simulink model "GIT_AUTO_Model_Example"  (R2019b)
settings: Solver=FixedStepDiscrete  StartTime=0.0  StopTime=10  FixedStep=0.01  RelTol=1e-3  EnableMultiTasking=on
InitFcn:
  | clear mex;
undefined symbols (not defined in the file): asbcbaseini_C, ibatini_C, k_icalpl_C, scsocini_C, stopengstmode_C, t_bmaxini_C, t_bminini_C, t_vminddstr_C, TSB_Coulomb_float, TSB_Dc_float, TSB_Pwr_float, TSB_R_float, TSB_Soc, TSB_Tbatt, TSB_Tbatt_float, TSB_value_float, TSB_Volt_float, v_bcini_C, v_bcmaxini_C
libraries: Utility_Block_Library x22, AMO_Block_Library x2
(part 4 of 5)

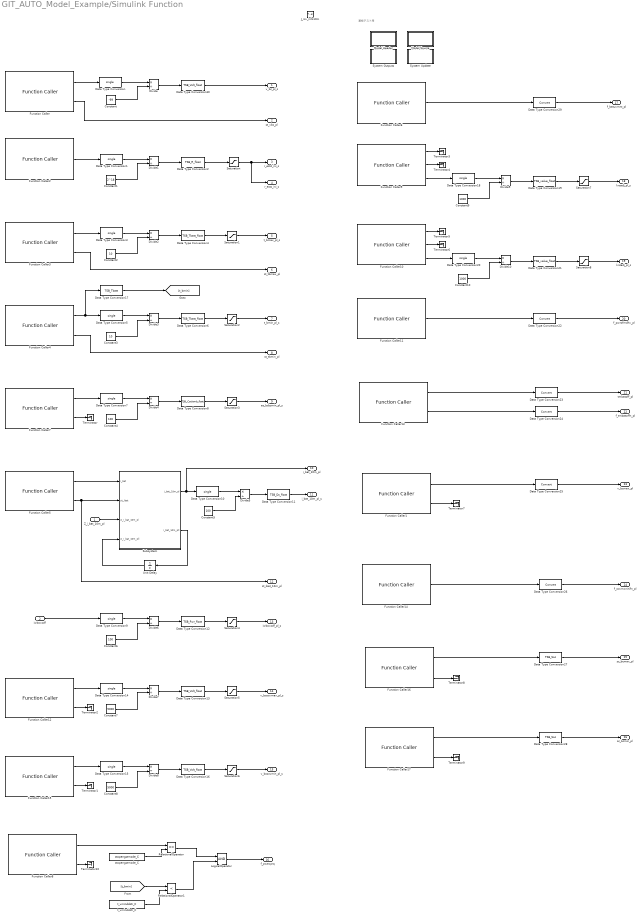
== system GIT_AUTO_Model_Example/Simulink Function ==
  note: 基板テスト用
  Z_i_bat_10m_pl : Inport  Tag=#AMO_Lib
      settings: AttributesFormatString=%<Tag>\n%<Description>\nSampleTime = %<SampleTime>
  iwboxcdf : Inport  Tag=#AMO_Lib  Port=2
      settings: AttributesFormatString=%<Tag>\n%<Description>\nSampleTime = %<SampleTime>
  J_rcv_info10m : TriggerPort  TriggerType=function-call  IsSimulinkFunction=on  FunctionName=J_rcv_info10m  VariantControl=(inherit)
  Constant : Constant  Tag=#AMO_Lib  Value=-99  OutDataTypeStr=single
      settings: AttributesFormatString=%<Tag>\nOutDataType = %<OutDataTypeStr>
  Constant1 : Constant  Tag=#AMO_Lib  Value=2^18  OutDataTypeStr=single
      settings: AttributesFormatString=%<Tag>\nOutDataType = %<OutDataTypeStr>
  Constant10 : Constant  Tag=#AMO_Lib  Value=1000  OutDataTypeStr=single
      settings: AttributesFormatString=%<Tag>\nOutDataType = %<OutDataTypeStr>
  Constant2 : Constant  Tag=#AMO_Lib  Value=10  OutDataTypeStr=single
      settings: AttributesFormatString=%<Tag>\nOutDataType = %<OutDataTypeStr>
  Constant3 : Constant  Tag=#AMO_Lib  Value=10  OutDataTypeStr=single
      settings: AttributesFormatString=%<Tag>\nOutDataType = %<OutDataTypeStr>
  Constant4 : Constant  Tag=#AMO_Lib  Value=100  OutDataTypeStr=single
      settings: AttributesFormatString=%<Tag>\nOutDataType = %<OutDataTypeStr>
  Constant5 : Constant  Tag=#AMO_Lib  Value=100  OutDataTypeStr=single
      settings: AttributesFormatString=%<Tag>\nOutDataType = %<OutDataTypeStr>
  Constant6 : Constant  Tag=#AMO_Lib  Value=100  OutDataTypeStr=single
      settings: AttributesFormatString=%<Tag>\nOutDataType = %<OutDataTypeStr>
  Constant7 : Constant  Tag=#AMO_Lib  Value=5000  OutDataTypeStr=single
      settings: AttributesFormatString=%<Tag>\nOutDataType = %<OutDataTypeStr>
  Constant8 : Constant  Tag=#AMO_Lib  Value=5000  OutDataTypeStr=single
      settings: AttributesFormatString=%<Tag>\nOutDataType = %<OutDataTypeStr>
  Constant9 : Constant  Tag=#AMO_Lib  Value=1000  OutDataTypeStr=single
      settings: AttributesFormatString=%<Tag>\nOutDataType = %<OutDataTypeStr>
  Data Type Conversion : DataTypeConversion  Tag=#AMO_Lib  OutMin=OutMin  OutMax=OutMax  OutDataTypeStr=single  ConvertRealWorld=Stored Integer (SI)  SampleTime=SampleTime  SaturateOnIntegerOverflow=on  RndMeth=Zero  mask{OutMin=[], OutMax=[], OutDataTypeStr=single, LockScale=off, ConvertRealWorld=Stored Integer (SI), RndMeth=Zero, SaturateOnIntegerOverflow=on, SampleTime=-1}
      mask prompts: OutMin "Simulink:blkprm_prompts:OutputDesignMin"; OutMax "Simulink:blkprm_prompts:OutputDesignMax"; OutDataTypeStr "Simulink:blkprm_prompts:OUTPUT_UNIFIEDDATATYPE"; LockScale "Simulink:blkprm_prompts:LockScale"; ConvertRealWorld "Simulink:blkprm_prompts:DtypeCnvInputOutputValue"; RndMeth "Simulink:blkprm_prompts:SPP_RndMeth_ID"; SaturateOnIntegerOverflow "Simulink:blkprm_prompts:AllBlksSaturate"; SampleTime "Simulink:blkprm_prompts:AllBlksSampleTime"
      mask help:
      | 入力を出力のデータ型とスケーリングに変換します。
      |
      | この変換には 2 つの目的があります。1 つは入力と出力の実際値を等しくすることです。もう 1 つは入力と出力の整数格納値を等しくすることです。オーバーフローと量子化誤差があると、この目的を完全に達成することができません。
      settings: AttributesFormatString=%<Tag>\nOutDataType = %<OutDataTypeStr>
      mask TypeOptions OutMin: OutMin
      mask TypeOptions OutMax: OutMax
      mask TypeOptions OutDataTypeStr: OutDataTypeStr
      mask TypeOptions LockScale: LockScale
      mask TypeOptions ConvertRealWorld: ConvertRealWorld
      mask TypeOptions RndMeth: RndMeth
      mask TypeOptions SaturateOnIntegerOverflow: SaturateOnIntegerOverflow
      mask TypeOptions SampleTime: SampleTime
      mask DialogControl OutMin Prompt: 出力の最小値:
      mask DialogControl OutMax Prompt: 出力の最大値:
      mask DialogControl OutDataTypeStr Prompt: 出力データ型:
      mask DialogControl LockScale Prompt: 固定小数点ツールによる変更に対して出力データ型の設定をロックする
      mask DialogControl ConvertRealWorld Prompt: 等価な値をもつ入力と出力:
      mask DialogControl RndMeth Prompt: 整数丸めモード:
      mask DialogControl SaturateOnIntegerOverflow Prompt: 整数オーバーフローで飽和
      mask DialogControl SampleTime Prompt: サンプル時間 (継承は -1):
  Data Type Conversion1 : DataTypeConversion  Tag=#AMO_Lib  OutMin=OutMin  OutMax=OutMax  OutDataTypeStr=single  ConvertRealWorld=Stored Integer (SI)  SampleTime=SampleTime  SaturateOnIntegerOverflow=on  RndMeth=Zero  mask{OutMin=[], OutMax=[], OutDataTypeStr=single, LockScale=off, ConvertRealWorld=Stored Integer (SI), RndMeth=Zero, SaturateOnIntegerOverflow=on, SampleTime=-1}
      mask prompts: OutMin "Simulink:blkprm_prompts:OutputDesignMin"; OutMax "Simulink:blkprm_prompts:OutputDesignMax"; OutDataTypeStr "Simulink:blkprm_prompts:OUTPUT_UNIFIEDDATATYPE"; LockScale "Simulink:blkprm_prompts:LockScale"; ConvertRealWorld "Simulink:blkprm_prompts:DtypeCnvInputOutputValue"; RndMeth "Simulink:blkprm_prompts:SPP_RndMeth_ID"; SaturateOnIntegerOverflow "Simulink:blkprm_prompts:AllBlksSaturate"; SampleTime "Simulink:blkprm_prompts:AllBlksSampleTime"
      mask help:
      | 入力を出力のデータ型とスケーリングに変換します。
      |
      | この変換には 2 つの目的があります。1 つは入力と出力の実際値を等しくすることです。もう 1 つは入力と出力の整数格納値を等しくすることです。オーバーフローと量子化誤差があると、この目的を完全に達成することができません。
      settings: AttributesFormatString=%<Tag>\nOutDataType = %<OutDataTypeStr>
      mask TypeOptions OutMin: OutMin
      mask TypeOptions OutMax: OutMax
      mask TypeOptions OutDataTypeStr: OutDataTypeStr
      mask TypeOptions LockScale: LockScale
      mask TypeOptions ConvertRealWorld: ConvertRealWorld
      mask TypeOptions RndMeth: RndMeth
      mask TypeOptions SaturateOnIntegerOverflow: SaturateOnIntegerOverflow
      mask TypeOptions SampleTime: SampleTime
      mask DialogControl OutMin Prompt: 出力の最小値:
      mask DialogControl OutMax Prompt: 出力の最大値:
      mask DialogControl OutDataTypeStr Prompt: 出力データ型:
      mask DialogControl LockScale Prompt: 固定小数点ツールによる変更に対して出力データ型の設定をロックする
      mask DialogControl ConvertRealWorld Prompt: 等価な値をもつ入力と出力:
      mask DialogControl RndMeth Prompt: 整数丸めモード:
      mask DialogControl SaturateOnIntegerOverflow Prompt: 整数オーバーフローで飽和
      mask DialogControl SampleTime Prompt: サンプル時間 (継承は -1):
  Data Type Conversion10 : DataTypeConversion  Tag=#AMO_Lib  OutMin=OutMin  OutMax=OutMax  OutDataTypeStr=single  ConvertRealWorld=Stored Integer (SI)  SampleTime=SampleTime  SaturateOnIntegerOverflow=on  RndMeth=Zero  mask{OutMin=[], OutMax=[], OutDataTypeStr=single, LockScale=off, ConvertRealWorld=Stored Integer (SI), RndMeth=Zero, SaturateOnIntegerOverflow=on, SampleTime=-1}
      mask prompts: OutMin "Simulink:blkprm_prompts:OutputDesignMin"; OutMax "Simulink:blkprm_prompts:OutputDesignMax"; OutDataTypeStr "Simulink:blkprm_prompts:OUTPUT_UNIFIEDDATATYPE"; LockScale "Simulink:blkprm_prompts:LockScale"; ConvertRealWorld "Simulink:blkprm_prompts:DtypeCnvInputOutputValue"; RndMeth "Simulink:blkprm_prompts:SPP_RndMeth_ID"; SaturateOnIntegerOverflow "Simulink:blkprm_prompts:AllBlksSaturate"; SampleTime "Simulink:blkprm_prompts:AllBlksSampleTime"
      mask help:
      | 入力を出力のデータ型とスケーリングに変換します。
      |
      | この変換には 2 つの目的があります。1 つは入力と出力の実際値を等しくすることです。もう 1 つは入力と出力の整数格納値を等しくすることです。オーバーフローと量子化誤差があると、この目的を完全に達成することができません。
      settings: AttributesFormatString=%<Tag>\nOutDataType = %<OutDataTypeStr>
      mask TypeOptions OutMin: OutMin
      mask TypeOptions OutMax: OutMax
      mask TypeOptions OutDataTypeStr: OutDataTypeStr
      mask TypeOptions LockScale: LockScale
      mask TypeOptions ConvertRealWorld: ConvertRealWorld
      mask TypeOptions RndMeth: RndMeth
      mask TypeOptions SaturateOnIntegerOverflow: SaturateOnIntegerOverflow
      mask TypeOptions SampleTime: SampleTime
      mask DialogControl OutMin Prompt: 出力の最小値:
      mask DialogControl OutMax Prompt: 出力の最大値:
      mask DialogControl OutDataTypeStr Prompt: 出力データ型:
      mask DialogControl LockScale Prompt: 固定小数点ツールによる変更に対して出力データ型の設定をロックする
      mask DialogControl ConvertRealWorld Prompt: 等価な値をもつ入力と出力:
      mask DialogControl RndMeth Prompt: 整数丸めモード:
      mask DialogControl SaturateOnIntegerOverflow Prompt: 整数オーバーフローで飽和
      mask DialogControl SampleTime Prompt: サンプル時間 (継承は -1):
  Data Type Conversion11 : DataTypeConversion  Tag=#AMO_Lib  OutMin=OutMin  OutMax=OutMax  OutDataTypeStr=TSB_Dc_float  SampleTime=SampleTime  SaturateOnIntegerOverflow=on  RndMeth=Zero  mask{OutMin=[], OutMax=[], OutDataTypeStr=TSB_Dc_float, LockScale=off, ConvertRealWorld=Real World Value (RWV), RndMeth=Zero, SaturateOnIntegerOverflow=on, SampleTime=-1}
      mask prompts: OutMin "Simulink:blkprm_prompts:OutputDesignMin"; OutMax "Simulink:blkprm_prompts:OutputDesignMax"; OutDataTypeStr "Simulink:blkprm_prompts:OUTPUT_UNIFIEDDATATYPE"; LockScale "Simulink:blkprm_prompts:LockScale"; ConvertRealWorld "Simulink:blkprm_prompts:DtypeCnvInputOutputValue"; RndMeth "Simulink:blkprm_prompts:SPP_RndMeth_ID"; SaturateOnIntegerOverflow "Simulink:blkprm_prompts:AllBlksSaturate"; SampleTime "Simulink:blkprm_prompts:AllBlksSampleTime"
      mask help:
      | 入力を出力のデータ型とスケーリングに変換します。
      |
      | この変換には 2 つの目的があります。1 つは入力と出力の実際値を等しくすることです。もう 1 つは入力と出力の整数格納値を等しくすることです。オーバーフローと量子化誤差があると、この目的を完全に達成することができません。
      settings: AttributesFormatString=%<Tag>\nOutDataType = %<OutDataTypeStr>
      mask TypeOptions OutMin: OutMin
      mask TypeOptions OutMax: OutMax
      mask TypeOptions OutDataTypeStr: OutDataTypeStr
      mask TypeOptions LockScale: LockScale
      mask TypeOptions ConvertRealWorld: ConvertRealWorld
      mask TypeOptions RndMeth: RndMeth
      mask TypeOptions SaturateOnIntegerOverflow: SaturateOnIntegerOverflow
      mask TypeOptions SampleTime: SampleTime
      mask DialogControl OutMin Prompt: 出力の最小値:
      mask DialogControl OutMax Prompt: 出力の最大値:
      mask DialogControl OutDataTypeStr Prompt: 出力データ型:
      mask DialogControl LockScale Prompt: 固定小数点ツールによる変更に対して出力データ型の設定をロックする
      mask DialogControl ConvertRealWorld Prompt: 等価な値をもつ入力と出力:
      mask DialogControl RndMeth Prompt: 整数丸めモード:
      mask DialogControl SaturateOnIntegerOverflow Prompt: 整数オーバーフローで飽和
      mask DialogControl SampleTime Prompt: サンプル時間 (継承は -1):
  Data Type Conversion12 : DataTypeConversion  Tag=#AMO_Lib  OutMin=OutMin  OutMax=OutMax  OutDataTypeStr=TSB_Pwr_float  SampleTime=SampleTime  SaturateOnIntegerOverflow=on  RndMeth=Zero  mask{OutMin=[], OutMax=[], OutDataTypeStr=TSB_Pwr_float, LockScale=off, ConvertRealWorld=Real World Value (RWV), RndMeth=Zero, SaturateOnIntegerOverflow=on, SampleTime=-1}
      mask prompts: OutMin "Simulink:blkprm_prompts:OutputDesignMin"; OutMax "Simulink:blkprm_prompts:OutputDesignMax"; OutDataTypeStr "Simulink:blkprm_prompts:OUTPUT_UNIFIEDDATATYPE"; LockScale "Simulink:blkprm_prompts:LockScale"; ConvertRealWorld "Simulink:blkprm_prompts:DtypeCnvInputOutputValue"; RndMeth "Simulink:blkprm_prompts:SPP_RndMeth_ID"; SaturateOnIntegerOverflow "Simulink:blkprm_prompts:AllBlksSaturate"; SampleTime "Simulink:blkprm_prompts:AllBlksSampleTime"
      mask help:
      | 入力を出力のデータ型とスケーリングに変換します。
      |
      | この変換には 2 つの目的があります。1 つは入力と出力の実際値を等しくすることです。もう 1 つは入力と出力の整数格納値を等しくすることです。オーバーフローと量子化誤差があると、この目的を完全に達成することができません。
      settings: AttributesFormatString=%<Tag>\nOutDataType = %<OutDataTypeStr>
      mask TypeOptions OutMin: OutMin
      mask TypeOptions OutMax: OutMax
      mask TypeOptions OutDataTypeStr: OutDataTypeStr
      mask TypeOptions LockScale: LockScale
      mask TypeOptions ConvertRealWorld: ConvertRealWorld
      mask TypeOptions RndMeth: RndMeth
      mask TypeOptions SaturateOnIntegerOverflow: SaturateOnIntegerOverflow
      mask TypeOptions SampleTime: SampleTime
      mask DialogControl OutMin Prompt: 出力の最小値:
      mask DialogControl OutMax Prompt: 出力の最大値:
      mask DialogControl OutDataTypeStr Prompt: 出力データ型:
      mask DialogControl LockScale Prompt: 固定小数点ツールによる変更に対して出力データ型の設定をロックする
      mask DialogControl ConvertRealWorld Prompt: 等価な値をもつ入力と出力:
      mask DialogControl RndMeth Prompt: 整数丸めモード:
      mask DialogControl SaturateOnIntegerOverflow Prompt: 整数オーバーフローで飽和
      mask DialogControl SampleTime Prompt: サンプル時間 (継承は -1):
  Data Type Conversion13 : DataTypeConversion  Tag=#AMO_Lib  OutMin=OutMin  OutMax=OutMax  OutDataTypeStr=TSB_Volt_float  SampleTime=SampleTime  SaturateOnIntegerOverflow=on  RndMeth=Zero  mask{OutMin=[], OutMax=[], OutDataTypeStr=TSB_Volt_float, LockScale=off, ConvertRealWorld=Real World Value (RWV), RndMeth=Zero, SaturateOnIntegerOverflow=on, SampleTime=-1}
      mask prompts: OutMin "Simulink:blkprm_prompts:OutputDesignMin"; OutMax "Simulink:blkprm_prompts:OutputDesignMax"; OutDataTypeStr "Simulink:blkprm_prompts:OUTPUT_UNIFIEDDATATYPE"; LockScale "Simulink:blkprm_prompts:LockScale"; ConvertRealWorld "Simulink:blkprm_prompts:DtypeCnvInputOutputValue"; RndMeth "Simulink:blkprm_prompts:SPP_RndMeth_ID"; SaturateOnIntegerOverflow "Simulink:blkprm_prompts:AllBlksSaturate"; SampleTime "Simulink:blkprm_prompts:AllBlksSampleTime"
      mask help:
      | 入力を出力のデータ型とスケーリングに変換します。
      |
      | この変換には 2 つの目的があります。1 つは入力と出力の実際値を等しくすることです。もう 1 つは入力と出力の整数格納値を等しくすることです。オーバーフローと量子化誤差があると、この目的を完全に達成することができません。
      settings: AttributesFormatString=%<Tag>\nOutDataType = %<OutDataTypeStr>
      mask TypeOptions OutMin: OutMin
      mask TypeOptions OutMax: OutMax
      mask TypeOptions OutDataTypeStr: OutDataTypeStr
      mask TypeOptions LockScale: LockScale
      mask TypeOptions ConvertRealWorld: ConvertRealWorld
      mask TypeOptions RndMeth: RndMeth
      mask TypeOptions SaturateOnIntegerOverflow: SaturateOnIntegerOverflow
      mask TypeOptions SampleTime: SampleTime
      mask DialogControl OutMin Prompt: 出力の最小値:
      mask DialogControl OutMax Prompt: 出力の最大値:
      mask DialogControl OutDataTypeStr Prompt: 出力データ型:
      mask DialogControl LockScale Prompt: 固定小数点ツールによる変更に対して出力データ型の設定をロックする
      mask DialogControl ConvertRealWorld Prompt: 等価な値をもつ入力と出力:
      mask DialogControl RndMeth Prompt: 整数丸めモード:
      mask DialogControl SaturateOnIntegerOverflow Prompt: 整数オーバーフローで飽和
      mask DialogControl SampleTime Prompt: サンプル時間 (継承は -1):
  Data Type Conversion14 : DataTypeConversion  Tag=#AMO_Lib  OutMin=OutMin  OutMax=OutMax  OutDataTypeStr=single  ConvertRealWorld=Stored Integer (SI)  SampleTime=SampleTime  SaturateOnIntegerOverflow=on  RndMeth=Zero  mask{OutMin=[], OutMax=[], OutDataTypeStr=single, LockScale=off, ConvertRealWorld=Stored Integer (SI), RndMeth=Zero, SaturateOnIntegerOverflow=on, SampleTime=-1}
      mask prompts: OutMin "Simulink:blkprm_prompts:OutputDesignMin"; OutMax "Simulink:blkprm_prompts:OutputDesignMax"; OutDataTypeStr "Simulink:blkprm_prompts:OUTPUT_UNIFIEDDATATYPE"; LockScale "Simulink:blkprm_prompts:LockScale"; ConvertRealWorld "Simulink:blkprm_prompts:DtypeCnvInputOutputValue"; RndMeth "Simulink:blkprm_prompts:SPP_RndMeth_ID"; SaturateOnIntegerOverflow "Simulink:blkprm_prompts:AllBlksSaturate"; SampleTime "Simulink:blkprm_prompts:AllBlksSampleTime"
      mask help:
      | 入力を出力のデータ型とスケーリングに変換します。
      |
      | この変換には 2 つの目的があります。1 つは入力と出力の実際値を等しくすることです。もう 1 つは入力と出力の整数格納値を等しくすることです。オーバーフローと量子化誤差があると、この目的を完全に達成することができません。
      settings: AttributesFormatString=%<Tag>\nOutDataType = %<OutDataTypeStr>
      mask TypeOptions OutMin: OutMin
      mask TypeOptions OutMax: OutMax
      mask TypeOptions OutDataTypeStr: OutDataTypeStr
      mask TypeOptions LockScale: LockScale
      mask TypeOptions ConvertRealWorld: ConvertRealWorld
      mask TypeOptions RndMeth: RndMeth
      mask TypeOptions SaturateOnIntegerOverflow: SaturateOnIntegerOverflow
      mask TypeOptions SampleTime: SampleTime
      mask DialogControl OutMin Prompt: 出力の最小値:
      mask DialogControl OutMax Prompt: 出力の最大値:
      mask DialogControl OutDataTypeStr Prompt: 出力データ型:
      mask DialogControl LockScale Prompt: 固定小数点ツールによる変更に対して出力データ型の設定をロックする
      mask DialogControl ConvertRealWorld Prompt: 等価な値をもつ入力と出力:
      mask DialogControl RndMeth Prompt: 整数丸めモード:
      mask DialogControl SaturateOnIntegerOverflow Prompt: 整数オーバーフローで飽和
      mask DialogControl SampleTime Prompt: サンプル時間 (継承は -1):
  Data Type Conversion15 : DataTypeConversion  Tag=#AMO_Lib  OutMin=OutMin  OutMax=OutMax  OutDataTypeStr=single  ConvertRealWorld=Stored Integer (SI)  SampleTime=SampleTime  SaturateOnIntegerOverflow=on  RndMeth=Zero  mask{OutMin=[], OutMax=[], OutDataTypeStr=single, LockScale=off, ConvertRealWorld=Stored Integer (SI), RndMeth=Zero, SaturateOnIntegerOverflow=on, SampleTime=-1}
      mask prompts: OutMin "Simulink:blkprm_prompts:OutputDesignMin"; OutMax "Simulink:blkprm_prompts:OutputDesignMax"; OutDataTypeStr "Simulink:blkprm_prompts:OUTPUT_UNIFIEDDATATYPE"; LockScale "Simulink:blkprm_prompts:LockScale"; ConvertRealWorld "Simulink:blkprm_prompts:DtypeCnvInputOutputValue"; RndMeth "Simulink:blkprm_prompts:SPP_RndMeth_ID"; SaturateOnIntegerOverflow "Simulink:blkprm_prompts:AllBlksSaturate"; SampleTime "Simulink:blkprm_prompts:AllBlksSampleTime"
      mask help:
      | 入力を出力のデータ型とスケーリングに変換します。
      |
      | この変換には 2 つの目的があります。1 つは入力と出力の実際値を等しくすることです。もう 1 つは入力と出力の整数格納値を等しくすることです。オーバーフローと量子化誤差があると、この目的を完全に達成することができません。
      settings: AttributesFormatString=%<Tag>\nOutDataType = %<OutDataTypeStr>
      mask TypeOptions OutMin: OutMin
      mask TypeOptions OutMax: OutMax
      mask TypeOptions OutDataTypeStr: OutDataTypeStr
      mask TypeOptions LockScale: LockScale
      mask TypeOptions ConvertRealWorld: ConvertRealWorld
      mask TypeOptions RndMeth: RndMeth
      mask TypeOptions SaturateOnIntegerOverflow: SaturateOnIntegerOverflow
      mask TypeOptions SampleTime: SampleTime
      mask DialogControl OutMin Prompt: 出力の最小値:
      mask DialogControl OutMax Prompt: 出力の最大値:
      mask DialogControl OutDataTypeStr Prompt: 出力データ型:
      mask DialogControl LockScale Prompt: 固定小数点ツールによる変更に対して出力データ型の設定をロックする
      mask DialogControl ConvertRealWorld Prompt: 等価な値をもつ入力と出力:
      mask DialogControl RndMeth Prompt: 整数丸めモード:
      mask DialogControl SaturateOnIntegerOverflow Prompt: 整数オーバーフローで飽和
      mask DialogControl SampleTime Prompt: サンプル時間 (継承は -1):
  Data Type Conversion16 : DataTypeConversion  Tag=#AMO_Lib  OutMin=OutMin  OutMax=OutMax  OutDataTypeStr=TSB_Volt_float  SampleTime=SampleTime  SaturateOnIntegerOverflow=on  RndMeth=Zero  mask{OutMin=[], OutMax=[], OutDataTypeStr=TSB_Volt_float, LockScale=off, ConvertRealWorld=Real World Value (RWV), RndMeth=Zero, SaturateOnIntegerOverflow=on, SampleTime=-1}
      mask prompts: OutMin "Simulink:blkprm_prompts:OutputDesignMin"; OutMax "Simulink:blkprm_prompts:OutputDesignMax"; OutDataTypeStr "Simulink:blkprm_prompts:OUTPUT_UNIFIEDDATATYPE"; LockScale "Simulink:blkprm_prompts:LockScale"; ConvertRealWorld "Simulink:blkprm_prompts:DtypeCnvInputOutputValue"; RndMeth "Simulink:blkprm_prompts:SPP_RndMeth_ID"; SaturateOnIntegerOverflow "Simulink:blkprm_prompts:AllBlksSaturate"; SampleTime "Simulink:blkprm_prompts:AllBlksSampleTime"
      mask help:
      | 入力を出力のデータ型とスケーリングに変換します。
      |
      | この変換には 2 つの目的があります。1 つは入力と出力の実際値を等しくすることです。もう 1 つは入力と出力の整数格納値を等しくすることです。オーバーフローと量子化誤差があると、この目的を完全に達成することができません。
      settings: AttributesFormatString=%<Tag>\nOutDataType = %<OutDataTypeStr>
      mask TypeOptions OutMin: OutMin
      mask TypeOptions OutMax: OutMax
      mask TypeOptions OutDataTypeStr: OutDataTypeStr
      mask TypeOptions LockScale: LockScale
      mask TypeOptions ConvertRealWorld: ConvertRealWorld
      mask TypeOptions RndMeth: RndMeth
      mask TypeOptions SaturateOnIntegerOverflow: SaturateOnIntegerOverflow
      mask TypeOptions SampleTime: SampleTime
      mask DialogControl OutMin Prompt: 出力の最小値:
      mask DialogControl OutMax Prompt: 出力の最大値:
      mask DialogControl OutDataTypeStr Prompt: 出力データ型:
      mask DialogControl LockScale Prompt: 固定小数点ツールによる変更に対して出力データ型の設定をロックする
      mask DialogControl ConvertRealWorld Prompt: 等価な値をもつ入力と出力:
      mask DialogControl RndMeth Prompt: 整数丸めモード:
      mask DialogControl SaturateOnIntegerOverflow Prompt: 整数オーバーフローで飽和
      mask DialogControl SampleTime Prompt: サンプル時間 (継承は -1):
  Data Type Conversion17 : DataTypeConversion  Tag=#AMO_Lib  OutMin=OutMin  OutMax=OutMax  OutDataTypeStr=TSB_Tbatt  ConvertRealWorld=Stored Integer (SI)  SampleTime=SampleTime  SaturateOnIntegerOverflow=on  RndMeth=Zero  mask{OutMin=[], OutMax=[], OutDataTypeStr=TSB_Tbatt, LockScale=off, ConvertRealWorld=Stored Integer (SI), RndMeth=Zero, SaturateOnIntegerOverflow=on, SampleTime=-1}
      mask prompts: OutMin "Simulink:blkprm_prompts:OutputDesignMin"; OutMax "Simulink:blkprm_prompts:OutputDesignMax"; OutDataTypeStr "Simulink:blkprm_prompts:OUTPUT_UNIFIEDDATATYPE"; LockScale "Simulink:blkprm_prompts:LockScale"; ConvertRealWorld "Simulink:blkprm_prompts:DtypeCnvInputOutputValue"; RndMeth "Simulink:blkprm_prompts:SPP_RndMeth_ID"; SaturateOnIntegerOverflow "Simulink:blkprm_prompts:AllBlksSaturate"; SampleTime "Simulink:blkprm_prompts:AllBlksSampleTime"
      mask help:
      | 入力を出力のデータ型とスケーリングに変換します。
      |
      | この変換には 2 つの目的があります。1 つは入力と出力の実際値を等しくすることです。もう 1 つは入力と出力の整数格納値を等しくすることです。オーバーフローと量子化誤差があると、この目的を完全に達成することができません。
      settings: AttributesFormatString=%<Tag>\nOutDataType = %<OutDataTypeStr>
      mask TypeOptions OutMin: OutMin
      mask TypeOptions OutMax: OutMax
      mask TypeOptions OutDataTypeStr: OutDataTypeStr
      mask TypeOptions LockScale: LockScale
      mask TypeOptions ConvertRealWorld: ConvertRealWorld
      mask TypeOptions RndMeth: RndMeth
      mask TypeOptions SaturateOnIntegerOverflow: SaturateOnIntegerOverflow
      mask TypeOptions SampleTime: SampleTime
      mask DialogControl OutMin Prompt: 出力の最小値:
      mask DialogControl OutMax Prompt: 出力の最大値:
      mask DialogControl OutDataTypeStr Prompt: 出力データ型:
      mask DialogControl LockScale Prompt: 固定小数点ツールによる変更に対して出力データ型の設定をロックする
      mask DialogControl ConvertRealWorld Prompt: 等価な値をもつ入力と出力:
      mask DialogControl RndMeth Prompt: 整数丸めモード:
      mask DialogControl SaturateOnIntegerOverflow Prompt: 整数オーバーフローで飽和
      mask DialogControl SampleTime Prompt: サンプル時間 (継承は -1):
  Data Type Conversion18 : DataTypeConversion  Tag=#AMO_Lib  OutMin=OutMin  OutMax=OutMax  OutDataTypeStr=single  ConvertRealWorld=Stored Integer (SI)  SampleTime=SampleTime  SaturateOnIntegerOverflow=on  RndMeth=Zero  mask{OutMin=[], OutMax=[], OutDataTypeStr=single, LockScale=off, ConvertRealWorld=Stored Integer (SI), RndMeth=Zero, SaturateOnIntegerOverflow=on, SampleTime=-1}
      mask prompts: OutMin "Simulink:blkprm_prompts:OutputDesignMin"; OutMax "Simulink:blkprm_prompts:OutputDesignMax"; OutDataTypeStr "Simulink:blkprm_prompts:OUTPUT_UNIFIEDDATATYPE"; LockScale "Simulink:blkprm_prompts:LockScale"; ConvertRealWorld "Simulink:blkprm_prompts:DtypeCnvInputOutputValue"; RndMeth "Simulink:blkprm_prompts:SPP_RndMeth_ID"; SaturateOnIntegerOverflow "Simulink:blkprm_prompts:AllBlksSaturate"; SampleTime "Simulink:blkprm_prompts:AllBlksSampleTime"
      mask help:
      | 入力を出力のデータ型とスケーリングに変換します。
      |
      | この変換には 2 つの目的があります。1 つは入力と出力の実際値を等しくすることです。もう 1 つは入力と出力の整数格納値を等しくすることです。オーバーフローと量子化誤差があると、この目的を完全に達成することができません。
      settings: AttributesFormatString=%<Tag>\nOutDataType = %<OutDataTypeStr>
      mask TypeOptions OutMin: OutMin
      mask TypeOptions OutMax: OutMax
      mask TypeOptions OutDataTypeStr: OutDataTypeStr
      mask TypeOptions LockScale: LockScale
      mask TypeOptions ConvertRealWorld: ConvertRealWorld
      mask TypeOptions RndMeth: RndMeth
      mask TypeOptions SaturateOnIntegerOverflow: SaturateOnIntegerOverflow
      mask TypeOptions SampleTime: SampleTime
      mask DialogControl OutMin Prompt: 出力の最小値:
      mask DialogControl OutMax Prompt: 出力の最大値:
      mask DialogControl OutDataTypeStr Prompt: 出力データ型:
      mask DialogControl LockScale Prompt: 固定小数点ツールによる変更に対して出力データ型の設定をロックする
      mask DialogControl ConvertRealWorld Prompt: 等価な値をもつ入力と出力:
      mask DialogControl RndMeth Prompt: 整数丸めモード:
      mask DialogControl SaturateOnIntegerOverflow Prompt: 整数オーバーフローで飽和
      mask DialogControl SampleTime Prompt: サンプル時間 (継承は -1):
  Data Type Conversion19 : DataTypeConversion  Tag=#AMO_Lib  OutMin=OutMin  OutMax=OutMax  OutDataTypeStr=TSB_value_float  SampleTime=SampleTime  SaturateOnIntegerOverflow=on  RndMeth=Zero  mask{OutMin=[], OutMax=[], OutDataTypeStr=TSB_value_float, LockScale=off, ConvertRealWorld=Real World Value (RWV), RndMeth=Zero, SaturateOnIntegerOverflow=on, SampleTime=-1}
      mask prompts: OutMin "Simulink:blkprm_prompts:OutputDesignMin"; OutMax "Simulink:blkprm_prompts:OutputDesignMax"; OutDataTypeStr "Simulink:blkprm_prompts:OUTPUT_UNIFIEDDATATYPE"; LockScale "Simulink:blkprm_prompts:LockScale"; ConvertRealWorld "Simulink:blkprm_prompts:DtypeCnvInputOutputValue"; RndMeth "Simulink:blkprm_prompts:SPP_RndMeth_ID"; SaturateOnIntegerOverflow "Simulink:blkprm_prompts:AllBlksSaturate"; SampleTime "Simulink:blkprm_prompts:AllBlksSampleTime"
      mask help:
      | 入力を出力のデータ型とスケーリングに変換します。
      |
      | この変換には 2 つの目的があります。1 つは入力と出力の実際値を等しくすることです。もう 1 つは入力と出力の整数格納値を等しくすることです。オーバーフローと量子化誤差があると、この目的を完全に達成することができません。
      settings: AttributesFormatString=%<Tag>\nOutDataType = %<OutDataTypeStr>
      mask TypeOptions OutMin: OutMin
      mask TypeOptions OutMax: OutMax
      mask TypeOptions OutDataTypeStr: OutDataTypeStr
      mask TypeOptions LockScale: LockScale
      mask TypeOptions ConvertRealWorld: ConvertRealWorld
      mask TypeOptions RndMeth: RndMeth
      mask TypeOptions SaturateOnIntegerOverflow: SaturateOnIntegerOverflow
      mask TypeOptions SampleTime: SampleTime
      mask DialogControl OutMin Prompt: 出力の最小値:
      mask DialogControl OutMax Prompt: 出力の最大値:
      mask DialogControl OutDataTypeStr Prompt: 出力データ型:
      mask DialogControl LockScale Prompt: 固定小数点ツールによる変更に対して出力データ型の設定をロックする
      mask DialogControl ConvertRealWorld Prompt: 等価な値をもつ入力と出力:
      mask DialogControl RndMeth Prompt: 整数丸めモード:
      mask DialogControl SaturateOnIntegerOverflow Prompt: 整数オーバーフローで飽和
      mask DialogControl SampleTime Prompt: サンプル時間 (継承は -1):
  Data Type Conversion2 : DataTypeConversion  Tag=#AMO_Lib  OutMin=OutMin  OutMax=OutMax  OutDataTypeStr=TSB_R_float  SampleTime=SampleTime  SaturateOnIntegerOverflow=on  RndMeth=Zero  mask{OutMin=[], OutMax=[], OutDataTypeStr=TSB_R_float, LockScale=off, ConvertRealWorld=Real World Value (RWV), RndMeth=Zero, SaturateOnIntegerOverflow=on, SampleTime=-1}
      mask prompts: OutMin "Simulink:blkprm_prompts:OutputDesignMin"; OutMax "Simulink:blkprm_prompts:OutputDesignMax"; OutDataTypeStr "Simulink:blkprm_prompts:OUTPUT_UNIFIEDDATATYPE"; LockScale "Simulink:blkprm_prompts:LockScale"; ConvertRealWorld "Simulink:blkprm_prompts:DtypeCnvInputOutputValue"; RndMeth "Simulink:blkprm_prompts:SPP_RndMeth_ID"; SaturateOnIntegerOverflow "Simulink:blkprm_prompts:AllBlksSaturate"; SampleTime "Simulink:blkprm_prompts:AllBlksSampleTime"
      mask help:
      | 入力を出力のデータ型とスケーリングに変換します。
      |
      | この変換には 2 つの目的があります。1 つは入力と出力の実際値を等しくすることです。もう 1 つは入力と出力の整数格納値を等しくすることです。オーバーフローと量子化誤差があると、この目的を完全に達成することができません。
      settings: AttributesFormatString=%<Tag>\nOutDataType = %<OutDataTypeStr>
      mask TypeOptions OutMin: OutMin
      mask TypeOptions OutMax: OutMax
      mask TypeOptions OutDataTypeStr: OutDataTypeStr
      mask TypeOptions LockScale: LockScale
      mask TypeOptions ConvertRealWorld: ConvertRealWorld
      mask TypeOptions RndMeth: RndMeth
      mask TypeOptions SaturateOnIntegerOverflow: SaturateOnIntegerOverflow
      mask TypeOptions SampleTime: SampleTime
      mask DialogControl OutMin Prompt: 出力の最小値:
      mask DialogControl OutMax Prompt: 出力の最大値:
      mask DialogControl OutDataTypeStr Prompt: 出力データ型:
      mask DialogControl LockScale Prompt: 固定小数点ツールによる変更に対して出力データ型の設定をロックする
      mask DialogControl ConvertRealWorld Prompt: 等価な値をもつ入力と出力:
      mask DialogControl RndMeth Prompt: 整数丸めモード:
      mask DialogControl SaturateOnIntegerOverflow Prompt: 整数オーバーフローで飽和
      mask DialogControl SampleTime Prompt: サンプル時間 (継承は -1):
  Data Type Conversion20 : DataTypeConversion  Tag=#AMO_Lib  OutMin=OutMin  OutMax=OutMax  OutDataTypeStr=single  ConvertRealWorld=Stored Integer (SI)  SampleTime=SampleTime  SaturateOnIntegerOverflow=on  RndMeth=Zero  mask{OutMin=[], OutMax=[], OutDataTypeStr=single, LockScale=off, ConvertRealWorld=Stored Integer (SI), RndMeth=Zero, SaturateOnIntegerOverflow=on, SampleTime=-1}
      mask prompts: OutMin "Simulink:blkprm_prompts:OutputDesignMin"; OutMax "Simulink:blkprm_prompts:OutputDesignMax"; OutDataTypeStr "Simulink:blkprm_prompts:OUTPUT_UNIFIEDDATATYPE"; LockScale "Simulink:blkprm_prompts:LockScale"; ConvertRealWorld "Simulink:blkprm_prompts:DtypeCnvInputOutputValue"; RndMeth "Simulink:blkprm_prompts:SPP_RndMeth_ID"; SaturateOnIntegerOverflow "Simulink:blkprm_prompts:AllBlksSaturate"; SampleTime "Simulink:blkprm_prompts:AllBlksSampleTime"
      mask help:
      | 入力を出力のデータ型とスケーリングに変換します。
      |
      | この変換には 2 つの目的があります。1 つは入力と出力の実際値を等しくすることです。もう 1 つは入力と出力の整数格納値を等しくすることです。オーバーフローと量子化誤差があると、この目的を完全に達成することができません。
      settings: AttributesFormatString=%<Tag>\nOutDataType = %<OutDataTypeStr>
      mask TypeOptions OutMin: OutMin
      mask TypeOptions OutMax: OutMax
      mask TypeOptions OutDataTypeStr: OutDataTypeStr
      mask TypeOptions LockScale: LockScale
      mask TypeOptions ConvertRealWorld: ConvertRealWorld
      mask TypeOptions RndMeth: RndMeth
      mask TypeOptions SaturateOnIntegerOverflow: SaturateOnIntegerOverflow
      mask TypeOptions SampleTime: SampleTime
      mask DialogControl OutMin Prompt: 出力の最小値:
      mask DialogControl OutMax Prompt: 出力の最大値:
      mask DialogControl OutDataTypeStr Prompt: 出力データ型:
      mask DialogControl LockScale Prompt: 固定小数点ツールによる変更に対して出力データ型の設定をロックする
      mask DialogControl ConvertRealWorld Prompt: 等価な値をもつ入力と出力:
      mask DialogControl RndMeth Prompt: 整数丸めモード:
      mask DialogControl SaturateOnIntegerOverflow Prompt: 整数オーバーフローで飽和
      mask DialogControl SampleTime Prompt: サンプル時間 (継承は -1):
  Data Type Conversion21 : DataTypeConversion  Tag=#AMO_Lib  OutMin=OutMin  OutMax=OutMax  OutDataTypeStr=TSB_value_float  SampleTime=SampleTime  SaturateOnIntegerOverflow=on  RndMeth=Zero  mask{OutMin=[], OutMax=[], OutDataTypeStr=TSB_value_float, LockScale=off, ConvertRealWorld=Real World Value (RWV), RndMeth=Zero, SaturateOnIntegerOverflow=on, SampleTime=-1}
      mask prompts: OutMin "Simulink:blkprm_prompts:OutputDesignMin"; OutMax "Simulink:blkprm_prompts:OutputDesignMax"; OutDataTypeStr "Simulink:blkprm_prompts:OUTPUT_UNIFIEDDATATYPE"; LockScale "Simulink:blkprm_prompts:LockScale"; ConvertRealWorld "Simulink:blkprm_prompts:DtypeCnvInputOutputValue"; RndMeth "Simulink:blkprm_prompts:SPP_RndMeth_ID"; SaturateOnIntegerOverflow "Simulink:blkprm_prompts:AllBlksSaturate"; SampleTime "Simulink:blkprm_prompts:AllBlksSampleTime"
      mask help:
      | 入力を出力のデータ型とスケーリングに変換します。
      |
      | この変換には 2 つの目的があります。1 つは入力と出力の実際値を等しくすることです。もう 1 つは入力と出力の整数格納値を等しくすることです。オーバーフローと量子化誤差があると、この目的を完全に達成することができません。
      settings: AttributesFormatString=%<Tag>\nOutDataType = %<OutDataTypeStr>
      mask TypeOptions OutMin: OutMin
      mask TypeOptions OutMax: OutMax
      mask TypeOptions OutDataTypeStr: OutDataTypeStr
      mask TypeOptions LockScale: LockScale
      mask TypeOptions ConvertRealWorld: ConvertRealWorld
      mask TypeOptions RndMeth: RndMeth
      mask TypeOptions SaturateOnIntegerOverflow: SaturateOnIntegerOverflow
      mask TypeOptions SampleTime: SampleTime
      mask DialogControl OutMin Prompt: 出力の最小値:
      mask DialogControl OutMax Prompt: 出力の最大値:
      mask DialogControl OutDataTypeStr Prompt: 出力データ型:
      mask DialogControl LockScale Prompt: 固定小数点ツールによる変更に対して出力データ型の設定をロックする
      mask DialogControl ConvertRealWorld Prompt: 等価な値をもつ入力と出力:
      mask DialogControl RndMeth Prompt: 整数丸めモード:
      mask DialogControl SaturateOnIntegerOverflow Prompt: 整数オーバーフローで飽和
      mask DialogControl SampleTime Prompt: サンプル時間 (継承は -1):
  Data Type Conversion22 : DataTypeConversion  Tag=#AMO_Lib  OutMin=OutMin  OutMax=OutMax  SampleTime=SampleTime  SaturateOnIntegerOverflow=on  RndMeth=Zero  mask{OutMin=[], OutMax=[], OutDataTypeStr=Inherit: Inherit via back propagation, LockScale=off, ConvertRealWorld=Real World Value (RWV), RndMeth=Zero, SaturateOnIntegerOverflow=on, SampleTime=-1}
      mask prompts: OutMin "Simulink:blkprm_prompts:OutputDesignMin"; OutMax "Simulink:blkprm_prompts:OutputDesignMax"; OutDataTypeStr "Simulink:blkprm_prompts:OUTPUT_UNIFIEDDATATYPE"; LockScale "Simulink:blkprm_prompts:LockScale"; ConvertRealWorld "Simulink:blkprm_prompts:DtypeCnvInputOutputValue"; RndMeth "Simulink:blkprm_prompts:SPP_RndMeth_ID"; SaturateOnIntegerOverflow "Simulink:blkprm_prompts:AllBlksSaturate"; SampleTime "Simulink:blkprm_prompts:AllBlksSampleTime"
      mask help:
      | 入力を出力のデータ型とスケーリングに変換します。
      |
      | この変換には 2 つの目的があります。1 つは入力と出力の実際値を等しくすることです。もう 1 つは入力と出力の整数格納値を等しくすることです。オーバーフローと量子化誤差があると、この目的を完全に達成することができません。
      settings: AttributesFormatString=%<Tag>\nOutDataType = %<OutDataTypeStr>
      mask TypeOptions OutMin: OutMin
      mask TypeOptions OutMax: OutMax
      mask TypeOptions OutDataTypeStr: OutDataTypeStr
      mask TypeOptions LockScale: LockScale
      mask TypeOptions ConvertRealWorld: ConvertRealWorld
      mask TypeOptions RndMeth: RndMeth
      mask TypeOptions SaturateOnIntegerOverflow: SaturateOnIntegerOverflow
      mask TypeOptions SampleTime: SampleTime
      mask DialogControl OutMin Prompt: 出力の最小値:
      mask DialogControl OutMax Prompt: 出力の最大値:
      mask DialogControl OutDataTypeStr Prompt: 出力データ型:
      mask DialogControl LockScale Prompt: 固定小数点ツールによる変更に対して出力データ型の設定をロックする
      mask DialogControl ConvertRealWorld Prompt: 等価な値をもつ入力と出力:
      mask DialogControl RndMeth Prompt: 整数丸めモード:
      mask DialogControl SaturateOnIntegerOverflow Prompt: 整数オーバーフローで飽和
      mask DialogControl SampleTime Prompt: サンプル時間 (継承は -1):
  Data Type Conversion23 : DataTypeConversion  Tag=#AMO_Lib  OutMin=OutMin  OutMax=OutMax  SampleTime=SampleTime  SaturateOnIntegerOverflow=on  RndMeth=Zero  mask{OutMin=[], OutMax=[], OutDataTypeStr=Inherit: Inherit via back propagation, LockScale=off, ConvertRealWorld=Real World Value (RWV), RndMeth=Zero, SaturateOnIntegerOverflow=on, SampleTime=-1}
      mask prompts: OutMin "Simulink:blkprm_prompts:OutputDesignMin"; OutMax "Simulink:blkprm_prompts:OutputDesignMax"; OutDataTypeStr "Simulink:blkprm_prompts:OUTPUT_UNIFIEDDATATYPE"; LockScale "Simulink:blkprm_prompts:LockScale"; ConvertRealWorld "Simulink:blkprm_prompts:DtypeCnvInputOutputValue"; RndMeth "Simulink:blkprm_prompts:SPP_RndMeth_ID"; SaturateOnIntegerOverflow "Simulink:blkprm_prompts:AllBlksSaturate"; SampleTime "Simulink:blkprm_prompts:AllBlksSampleTime"
      mask help:
      | 入力を出力のデータ型とスケーリングに変換します。
      |
      | この変換には 2 つの目的があります。1 つは入力と出力の実際値を等しくすることです。もう 1 つは入力と出力の整数格納値を等しくすることです。オーバーフローと量子化誤差があると、この目的を完全に達成することができません。
      settings: AttributesFormatString=%<Tag>\nOutDataType = %<OutDataTypeStr>
      mask TypeOptions OutMin: OutMin
      mask TypeOptions OutMax: OutMax
      mask TypeOptions OutDataTypeStr: OutDataTypeStr
      mask TypeOptions LockScale: LockScale
      mask TypeOptions ConvertRealWorld: ConvertRealWorld
      mask TypeOptions RndMeth: RndMeth
      mask TypeOptions SaturateOnIntegerOverflow: SaturateOnIntegerOverflow
      mask TypeOptions SampleTime: SampleTime
      mask DialogControl OutMin Prompt: 出力の最小値:
      mask DialogControl OutMax Prompt: 出力の最大値:
      mask DialogControl OutDataTypeStr Prompt: 出力データ型:
      mask DialogControl LockScale Prompt: 固定小数点ツールによる変更に対して出力データ型の設定をロックする
      mask DialogControl ConvertRealWorld Prompt: 等価な値をもつ入力と出力:
      mask DialogControl RndMeth Prompt: 整数丸めモード:
      mask DialogControl SaturateOnIntegerOverflow Prompt: 整数オーバーフローで飽和
      mask DialogControl SampleTime Prompt: サンプル時間 (継承は -1):
  Data Type Conversion24 : DataTypeConversion  Tag=#AMO_Lib  OutMin=OutMin  OutMax=OutMax  SampleTime=SampleTime  SaturateOnIntegerOverflow=on  RndMeth=Zero  mask{OutMin=[], OutMax=[], OutDataTypeStr=Inherit: Inherit via back propagation, LockScale=off, ConvertRealWorld=Real World Value (RWV), RndMeth=Zero, SaturateOnIntegerOverflow=on, SampleTime=-1}
      mask prompts: OutMin "Simulink:blkprm_prompts:OutputDesignMin"; OutMax "Simulink:blkprm_prompts:OutputDesignMax"; OutDataTypeStr "Simulink:blkprm_prompts:OUTPUT_UNIFIEDDATATYPE"; LockScale "Simulink:blkprm_prompts:LockScale"; ConvertRealWorld "Simulink:blkprm_prompts:DtypeCnvInputOutputValue"; RndMeth "Simulink:blkprm_prompts:SPP_RndMeth_ID"; SaturateOnIntegerOverflow "Simulink:blkprm_prompts:AllBlksSaturate"; SampleTime "Simulink:blkprm_prompts:AllBlksSampleTime"
      mask help:
      | 入力を出力のデータ型とスケーリングに変換します。
      |
      | この変換には 2 つの目的があります。1 つは入力と出力の実際値を等しくすることです。もう 1 つは入力と出力の整数格納値を等しくすることです。オーバーフローと量子化誤差があると、この目的を完全に達成することができません。
      settings: AttributesFormatString=%<Tag>\nOutDataType = %<OutDataTypeStr>
      mask TypeOptions OutMin: OutMin
      mask TypeOptions OutMax: OutMax
      mask TypeOptions OutDataTypeStr: OutDataTypeStr
      mask TypeOptions LockScale: LockScale
      mask TypeOptions ConvertRealWorld: ConvertRealWorld
      mask TypeOptions RndMeth: RndMeth
      mask TypeOptions SaturateOnIntegerOverflow: SaturateOnIntegerOverflow
      mask TypeOptions SampleTime: SampleTime
      mask DialogControl OutMin Prompt: 出力の最小値:
      mask DialogControl OutMax Prompt: 出力の最大値:
      mask DialogControl OutDataTypeStr Prompt: 出力データ型:
      mask DialogControl LockScale Prompt: 固定小数点ツールによる変更に対して出力データ型の設定をロックする
      mask DialogControl ConvertRealWorld Prompt: 等価な値をもつ入力と出力:
      mask DialogControl RndMeth Prompt: 整数丸めモード:
      mask DialogControl SaturateOnIntegerOverflow Prompt: 整数オーバーフローで飽和
      mask DialogControl SampleTime Prompt: サンプル時間 (継承は -1):
  Data Type Conversion25 : DataTypeConversion  Tag=#AMO_Lib  OutMin=OutMin  OutMax=OutMax  ConvertRealWorld=Stored Integer (SI)  SampleTime=SampleTime  SaturateOnIntegerOverflow=on  RndMeth=Zero  mask{OutMin=[], OutMax=[], OutDataTypeStr=Inherit: Inherit via back propagation, LockScale=off, ConvertRealWorld=Stored Integer (SI), RndMeth=Zero, SaturateOnIntegerOverflow=on, SampleTime=-1}
      mask prompts: OutMin "Simulink:blkprm_prompts:OutputDesignMin"; OutMax "Simulink:blkprm_prompts:OutputDesignMax"; OutDataTypeStr "Simulink:blkprm_prompts:OUTPUT_UNIFIEDDATATYPE"; LockScale "Simulink:blkprm_prompts:LockScale"; ConvertRealWorld "Simulink:blkprm_prompts:DtypeCnvInputOutputValue"; RndMeth "Simulink:blkprm_prompts:SPP_RndMeth_ID"; SaturateOnIntegerOverflow "Simulink:blkprm_prompts:AllBlksSaturate"; SampleTime "Simulink:blkprm_prompts:AllBlksSampleTime"
      mask help:
      | 入力を出力のデータ型とスケーリングに変換します。
      |
      | この変換には 2 つの目的があります。1 つは入力と出力の実際値を等しくすることです。もう 1 つは入力と出力の整数格納値を等しくすることです。オーバーフローと量子化誤差があると、この目的を完全に達成することができません。
      settings: AttributesFormatString=%<Tag>\nOutDataType = %<OutDataTypeStr>
      mask TypeOptions OutMin: OutMin
      mask TypeOptions OutMax: OutMax
      mask TypeOptions OutDataTypeStr: OutDataTypeStr
      mask TypeOptions LockScale: LockScale
      mask TypeOptions ConvertRealWorld: ConvertRealWorld
      mask TypeOptions RndMeth: RndMeth
      mask TypeOptions SaturateOnIntegerOverflow: SaturateOnIntegerOverflow
      mask TypeOptions SampleTime: SampleTime
      mask DialogControl OutMin Prompt: 出力の最小値:
      mask DialogControl OutMax Prompt: 出力の最大値:
      mask DialogControl OutDataTypeStr Prompt: 出力データ型:
      mask DialogControl LockScale Prompt: 固定小数点ツールによる変更に対して出力データ型の設定をロックする
      mask DialogControl ConvertRealWorld Prompt: 等価な値をもつ入力と出力:
      mask DialogControl RndMeth Prompt: 整数丸めモード:
      mask DialogControl SaturateOnIntegerOverflow Prompt: 整数オーバーフローで飽和
      mask DialogControl SampleTime Prompt: サンプル時間 (継承は -1):
  Data Type Conversion26 : DataTypeConversion  Tag=#AMO_Lib  OutMin=OutMin  OutMax=OutMax  SampleTime=SampleTime  SaturateOnIntegerOverflow=on  RndMeth=Zero  mask{OutMin=[], OutMax=[], OutDataTypeStr=Inherit: Inherit via back propagation, LockScale=off, ConvertRealWorld=Real World Value (RWV), RndMeth=Zero, SaturateOnIntegerOverflow=on, SampleTime=-1}
      mask prompts: OutMin "Simulink:blkprm_prompts:OutputDesignMin"; OutMax "Simulink:blkprm_prompts:OutputDesignMax"; OutDataTypeStr "Simulink:blkprm_prompts:OUTPUT_UNIFIEDDATATYPE"; LockScale "Simulink:blkprm_prompts:LockScale"; ConvertRealWorld "Simulink:blkprm_prompts:DtypeCnvInputOutputValue"; RndMeth "Simulink:blkprm_prompts:SPP_RndMeth_ID"; SaturateOnIntegerOverflow "Simulink:blkprm_prompts:AllBlksSaturate"; SampleTime "Simulink:blkprm_prompts:AllBlksSampleTime"
      mask help:
      | 入力を出力のデータ型とスケーリングに変換します。
      |
      | この変換には 2 つの目的があります。1 つは入力と出力の実際値を等しくすることです。もう 1 つは入力と出力の整数格納値を等しくすることです。オーバーフローと量子化誤差があると、この目的を完全に達成することができません。
      settings: AttributesFormatString=%<Tag>\nOutDataType = %<OutDataTypeStr>
      mask TypeOptions OutMin: OutMin
      mask TypeOptions OutMax: OutMax
      mask TypeOptions OutDataTypeStr: OutDataTypeStr
      mask TypeOptions LockScale: LockScale
      mask TypeOptions ConvertRealWorld: ConvertRealWorld
      mask TypeOptions RndMeth: RndMeth
      mask TypeOptions SaturateOnIntegerOverflow: SaturateOnIntegerOverflow
      mask TypeOptions SampleTime: SampleTime
      mask DialogControl OutMin Prompt: 出力の最小値:
      mask DialogControl OutMax Prompt: 出力の最大値:
      mask DialogControl OutDataTypeStr Prompt: 出力データ型:
      mask DialogControl LockScale Prompt: 固定小数点ツールによる変更に対して出力データ型の設定をロックする
      mask DialogControl ConvertRealWorld Prompt: 等価な値をもつ入力と出力:
      mask DialogControl RndMeth Prompt: 整数丸めモード:
      mask DialogControl SaturateOnIntegerOverflow Prompt: 整数オーバーフローで飽和
      mask DialogControl SampleTime Prompt: サンプル時間 (継承は -1):
  Data Type Conversion27 : DataTypeConversion  Tag=#AMO_Lib  OutMin=OutMin  OutMax=OutMax  OutDataTypeStr=TSB_Soc  ConvertRealWorld=Stored Integer (SI)  SampleTime=SampleTime  SaturateOnIntegerOverflow=on  RndMeth=Zero  mask{OutMin=[], OutMax=[], OutDataTypeStr=TSB_Soc, LockScale=off, ConvertRealWorld=Stored Integer (SI), RndMeth=Zero, SaturateOnIntegerOverflow=on, SampleTime=-1}
      mask prompts: OutMin "Simulink:blkprm_prompts:OutputDesignMin"; OutMax "Simulink:blkprm_prompts:OutputDesignMax"; OutDataTypeStr "Simulink:blkprm_prompts:OUTPUT_UNIFIEDDATATYPE"; LockScale "Simulink:blkprm_prompts:LockScale"; ConvertRealWorld "Simulink:blkprm_prompts:DtypeCnvInputOutputValue"; RndMeth "Simulink:blkprm_prompts:SPP_RndMeth_ID"; SaturateOnIntegerOverflow "Simulink:blkprm_prompts:AllBlksSaturate"; SampleTime "Simulink:blkprm_prompts:AllBlksSampleTime"
      mask help:
      | 入力を出力のデータ型とスケーリングに変換します。
      |
      | この変換には 2 つの目的があります。1 つは入力と出力の実際値を等しくすることです。もう 1 つは入力と出力の整数格納値を等しくすることです。オーバーフローと量子化誤差があると、この目的を完全に達成することができません。
      settings: AttributesFormatString=%<Tag>\nOutDataType = %<OutDataTypeStr>
      mask TypeOptions OutMin: OutMin
      mask TypeOptions OutMax: OutMax
      mask TypeOptions OutDataTypeStr: OutDataTypeStr
      mask TypeOptions LockScale: LockScale
      mask TypeOptions ConvertRealWorld: ConvertRealWorld
      mask TypeOptions RndMeth: RndMeth
      mask TypeOptions SaturateOnIntegerOverflow: SaturateOnIntegerOverflow
      mask TypeOptions SampleTime: SampleTime
      mask DialogControl OutMin Prompt: 出力の最小値:
      mask DialogControl OutMax Prompt: 出力の最大値:
      mask DialogControl OutDataTypeStr Prompt: 出力データ型:
      mask DialogControl LockScale Prompt: 固定小数点ツールによる変更に対して出力データ型の設定をロックする
      mask DialogControl ConvertRealWorld Prompt: 等価な値をもつ入力と出力:
      mask DialogControl RndMeth Prompt: 整数丸めモード:
      mask DialogControl SaturateOnIntegerOverflow Prompt: 整数オーバーフローで飽和
      mask DialogControl SampleTime Prompt: サンプル時間 (継承は -1):
  Data Type Conversion28 : DataTypeConversion  Tag=#AMO_Lib  OutMin=OutMin  OutMax=OutMax  OutDataTypeStr=TSB_Soc  ConvertRealWorld=Stored Integer (SI)  SampleTime=SampleTime  SaturateOnIntegerOverflow=on  RndMeth=Zero  mask{OutMin=[], OutMax=[], OutDataTypeStr=TSB_Soc, LockScale=off, ConvertRealWorld=Stored Integer (SI), RndMeth=Zero, SaturateOnIntegerOverflow=on, SampleTime=-1}
      mask prompts: OutMin "Simulink:blkprm_prompts:OutputDesignMin"; OutMax "Simulink:blkprm_prompts:OutputDesignMax"; OutDataTypeStr "Simulink:blkprm_prompts:OUTPUT_UNIFIEDDATATYPE"; LockScale "Simulink:blkprm_prompts:LockScale"; ConvertRealWorld "Simulink:blkprm_prompts:DtypeCnvInputOutputValue"; RndMeth "Simulink:blkprm_prompts:SPP_RndMeth_ID"; SaturateOnIntegerOverflow "Simulink:blkprm_prompts:AllBlksSaturate"; SampleTime "Simulink:blkprm_prompts:AllBlksSampleTime"
      mask help:
      | 入力を出力のデータ型とスケーリングに変換します。
      |
      | この変換には 2 つの目的があります。1 つは入力と出力の実際値を等しくすることです。もう 1 つは入力と出力の整数格納値を等しくすることです。オーバーフローと量子化誤差があると、この目的を完全に達成することができません。
      settings: AttributesFormatString=%<Tag>\nOutDataType = %<OutDataTypeStr>
      mask TypeOptions OutMin: OutMin
      mask TypeOptions OutMax: OutMax
      mask TypeOptions OutDataTypeStr: OutDataTypeStr
      mask TypeOptions LockScale: LockScale
      mask TypeOptions ConvertRealWorld: ConvertRealWorld
      mask TypeOptions RndMeth: RndMeth
      mask TypeOptions SaturateOnIntegerOverflow: SaturateOnIntegerOverflow
      mask TypeOptions SampleTime: SampleTime
      mask DialogControl OutMin Prompt: 出力の最小値:
      mask DialogControl OutMax Prompt: 出力の最大値:
      mask DialogControl OutDataTypeStr Prompt: 出力データ型:
      mask DialogControl LockScale Prompt: 固定小数点ツールによる変更に対して出力データ型の設定をロックする
      mask DialogControl ConvertRealWorld Prompt: 等価な値をもつ入力と出力:
      mask DialogControl RndMeth Prompt: 整数丸めモード:
      mask DialogControl SaturateOnIntegerOverflow Prompt: 整数オーバーフローで飽和
      mask DialogControl SampleTime Prompt: サンプル時間 (継承は -1):
  Data Type Conversion29 : DataTypeConversion  Tag=#AMO_Lib  OutMin=OutMin  OutMax=OutMax  SampleTime=SampleTime  SaturateOnIntegerOverflow=on  RndMeth=Zero  mask{OutMin=[], OutMax=[], OutDataTypeStr=Inherit: Inherit via back propagation, LockScale=off, ConvertRealWorld=Real World Value (RWV), RndMeth=Zero, SaturateOnIntegerOverflow=on, SampleTime=-1}
      mask prompts: OutMin "Simulink:blkprm_prompts:OutputDesignMin"; OutMax "Simulink:blkprm_prompts:OutputDesignMax"; OutDataTypeStr "Simulink:blkprm_prompts:OUTPUT_UNIFIEDDATATYPE"; LockScale "Simulink:blkprm_prompts:LockScale"; ConvertRealWorld "Simulink:blkprm_prompts:DtypeCnvInputOutputValue"; RndMeth "Simulink:blkprm_prompts:SPP_RndMeth_ID"; SaturateOnIntegerOverflow "Simulink:blkprm_prompts:AllBlksSaturate"; SampleTime "Simulink:blkprm_prompts:AllBlksSampleTime"
      mask help:
      | 入力を出力のデータ型とスケーリングに変換します。
      |
      | この変換には 2 つの目的があります。1 つは入力と出力の実際値を等しくすることです。もう 1 つは入力と出力の整数格納値を等しくすることです。オーバーフローと量子化誤差があると、この目的を完全に達成することができません。
      settings: AttributesFormatString=%<Tag>\nOutDataType = %<OutDataTypeStr>
      mask TypeOptions OutMin: OutMin
      mask TypeOptions OutMax: OutMax
      mask TypeOptions OutDataTypeStr: OutDataTypeStr
      mask TypeOptions LockScale: LockScale
      mask TypeOptions ConvertRealWorld: ConvertRealWorld
      mask TypeOptions RndMeth: RndMeth
      mask TypeOptions SaturateOnIntegerOverflow: SaturateOnIntegerOverflow
      mask TypeOptions SampleTime: SampleTime
      mask DialogControl OutMin Prompt: 出力の最小値:
      mask DialogControl OutMax Prompt: 出力の最大値:
      mask DialogControl OutDataTypeStr Prompt: 出力データ型:
      mask DialogControl LockScale Prompt: 固定小数点ツールによる変更に対して出力データ型の設定をロックする
      mask DialogControl ConvertRealWorld Prompt: 等価な値をもつ入力と出力:
      mask DialogControl RndMeth Prompt: 整数丸めモード:
      mask DialogControl SaturateOnIntegerOverflow Prompt: 整数オーバーフローで飽和
      mask DialogControl SampleTime Prompt: サンプル時間 (継承は -1):
  Data Type Conversion3 : DataTypeConversion  Tag=#AMO_Lib  OutMin=OutMin  OutMax=OutMax  OutDataTypeStr=single  ConvertRealWorld=Stored Integer (SI)  SampleTime=SampleTime  SaturateOnIntegerOverflow=on  RndMeth=Zero  mask{OutMin=[], OutMax=[], OutDataTypeStr=single, LockScale=off, ConvertRealWorld=Stored Integer (SI), RndMeth=Zero, SaturateOnIntegerOverflow=on, SampleTime=-1}
      mask prompts: OutMin "Simulink:blkprm_prompts:OutputDesignMin"; OutMax "Simulink:blkprm_prompts:OutputDesignMax"; OutDataTypeStr "Simulink:blkprm_prompts:OUTPUT_UNIFIEDDATATYPE"; LockScale "Simulink:blkprm_prompts:LockScale"; ConvertRealWorld "Simulink:blkprm_prompts:DtypeCnvInputOutputValue"; RndMeth "Simulink:blkprm_prompts:SPP_RndMeth_ID"; SaturateOnIntegerOverflow "Simulink:blkprm_prompts:AllBlksSaturate"; SampleTime "Simulink:blkprm_prompts:AllBlksSampleTime"
      mask help:
      | 入力を出力のデータ型とスケーリングに変換します。
      |
      | この変換には 2 つの目的があります。1 つは入力と出力の実際値を等しくすることです。もう 1 つは入力と出力の整数格納値を等しくすることです。オーバーフローと量子化誤差があると、この目的を完全に達成することができません。
      settings: AttributesFormatString=%<Tag>\nOutDataType = %<OutDataTypeStr>
      mask TypeOptions OutMin: OutMin
      mask TypeOptions OutMax: OutMax
      mask TypeOptions OutDataTypeStr: OutDataTypeStr
      mask TypeOptions LockScale: LockScale
      mask TypeOptions ConvertRealWorld: ConvertRealWorld
      mask TypeOptions RndMeth: RndMeth
      mask TypeOptions SaturateOnIntegerOverflow: SaturateOnIntegerOverflow
      mask TypeOptions SampleTime: SampleTime
      mask DialogControl OutMin Prompt: 出力の最小値:
      mask DialogControl OutMax Prompt: 出力の最大値:
      mask DialogControl OutDataTypeStr Prompt: 出力データ型:
      mask DialogControl LockScale Prompt: 固定小数点ツールによる変更に対して出力データ型の設定をロックする
      mask DialogControl ConvertRealWorld Prompt: 等価な値をもつ入力と出力:
      mask DialogControl RndMeth Prompt: 整数丸めモード:
      mask DialogControl SaturateOnIntegerOverflow Prompt: 整数オーバーフローで飽和
      mask DialogControl SampleTime Prompt: サンプル時間 (継承は -1):
  Data Type Conversion30 : DataTypeConversion  Tag=#AMO_Lib  OutMin=OutMin  OutMax=OutMax  OutDataTypeStr=TSB_Volt_float  SampleTime=SampleTime  SaturateOnIntegerOverflow=on  RndMeth=Zero  mask{OutMin=[], OutMax=[], OutDataTypeStr=TSB_Volt_float, LockScale=off, ConvertRealWorld=Real World Value (RWV), RndMeth=Zero, SaturateOnIntegerOverflow=on, SampleTime=-1}
      mask prompts: OutMin "Simulink:blkprm_prompts:OutputDesignMin"; OutMax "Simulink:blkprm_prompts:OutputDesignMax"; OutDataTypeStr "Simulink:blkprm_prompts:OUTPUT_UNIFIEDDATATYPE"; LockScale "Simulink:blkprm_prompts:LockScale"; ConvertRealWorld "Simulink:blkprm_prompts:DtypeCnvInputOutputValue"; RndMeth "Simulink:blkprm_prompts:SPP_RndMeth_ID"; SaturateOnIntegerOverflow "Simulink:blkprm_prompts:AllBlksSaturate"; SampleTime "Simulink:blkprm_prompts:AllBlksSampleTime"
      mask help:
      | 入力を出力のデータ型とスケーリングに変換します。
      |
      | この変換には 2 つの目的があります。1 つは入力と出力の実際値を等しくすることです。もう 1 つは入力と出力の整数格納値を等しくすることです。オーバーフローと量子化誤差があると、この目的を完全に達成することができません。
      settings: AttributesFormatString=%<Tag>\nOutDataType = %<OutDataTypeStr>
      mask TypeOptions OutMin: OutMin
      mask TypeOptions OutMax: OutMax
      mask TypeOptions OutDataTypeStr: OutDataTypeStr
      mask TypeOptions LockScale: LockScale
      mask TypeOptions ConvertRealWorld: ConvertRealWorld
      mask TypeOptions RndMeth: RndMeth
      mask TypeOptions SaturateOnIntegerOverflow: SaturateOnIntegerOverflow
      mask TypeOptions SampleTime: SampleTime
      mask DialogControl OutMin Prompt: 出力の最小値:
      mask DialogControl OutMax Prompt: 出力の最大値:
      mask DialogControl OutDataTypeStr Prompt: 出力データ型:
      mask DialogControl LockScale Prompt: 固定小数点ツールによる変更に対して出力データ型の設定をロックする
      mask DialogControl ConvertRealWorld Prompt: 等価な値をもつ入力と出力:
      mask DialogControl RndMeth Prompt: 整数丸めモード:
      mask DialogControl SaturateOnIntegerOverflow Prompt: 整数オーバーフローで飽和
      mask DialogControl SampleTime Prompt: サンプル時間 (継承は -1):
  Data Type Conversion4 : DataTypeConversion  Tag=#AMO_Lib  OutMin=OutMin  OutMax=OutMax  OutDataTypeStr=TSB_Tbatt_float  SampleTime=SampleTime  SaturateOnIntegerOverflow=on  RndMeth=Zero  mask{OutMin=[], OutMax=[], OutDataTypeStr=TSB_Tbatt_float, LockScale=off, ConvertRealWorld=Real World Value (RWV), RndMeth=Zero, SaturateOnIntegerOverflow=on, SampleTime=-1}
      mask prompts: OutMin "Simulink:blkprm_prompts:OutputDesignMin"; OutMax "Simulink:blkprm_prompts:OutputDesignMax"; OutDataTypeStr "Simulink:blkprm_prompts:OUTPUT_UNIFIEDDATATYPE"; LockScale "Simulink:blkprm_prompts:LockScale"; ConvertRealWorld "Simulink:blkprm_prompts:DtypeCnvInputOutputValue"; RndMeth "Simulink:blkprm_prompts:SPP_RndMeth_ID"; SaturateOnIntegerOverflow "Simulink:blkprm_prompts:AllBlksSaturate"; SampleTime "Simulink:blkprm_prompts:AllBlksSampleTime"
      mask help:
      | 入力を出力のデータ型とスケーリングに変換します。
      |
      | この変換には 2 つの目的があります。1 つは入力と出力の実際値を等しくすることです。もう 1 つは入力と出力の整数格納値を等しくすることです。オーバーフローと量子化誤差があると、この目的を完全に達成することができません。
      settings: AttributesFormatString=%<Tag>\nOutDataType = %<OutDataTypeStr>
      mask TypeOptions OutMin: OutMin
      mask TypeOptions OutMax: OutMax
      mask TypeOptions OutDataTypeStr: OutDataTypeStr
      mask TypeOptions LockScale: LockScale
      mask TypeOptions ConvertRealWorld: ConvertRealWorld
      mask TypeOptions RndMeth: RndMeth
      mask TypeOptions SaturateOnIntegerOverflow: SaturateOnIntegerOverflow
      mask TypeOptions SampleTime: SampleTime
      mask DialogControl OutMin Prompt: 出力の最小値:
      mask DialogControl OutMax Prompt: 出力の最大値:
      mask DialogControl OutDataTypeStr Prompt: 出力データ型:
      mask DialogControl LockScale Prompt: 固定小数点ツールによる変更に対して出力データ型の設定をロックする
      mask DialogControl ConvertRealWorld Prompt: 等価な値をもつ入力と出力:
      mask DialogControl RndMeth Prompt: 整数丸めモード:
      mask DialogControl SaturateOnIntegerOverflow Prompt: 整数オーバーフローで飽和
      mask DialogControl SampleTime Prompt: サンプル時間 (継承は -1):
  Data Type Conversion5 : DataTypeConversion  Tag=#AMO_Lib  OutMin=OutMin  OutMax=OutMax  OutDataTypeStr=single  ConvertRealWorld=Stored Integer (SI)  SampleTime=SampleTime  SaturateOnIntegerOverflow=on  RndMeth=Zero  mask{OutMin=[], OutMax=[], OutDataTypeStr=single, LockScale=off, ConvertRealWorld=Stored Integer (SI), RndMeth=Zero, SaturateOnIntegerOverflow=on, SampleTime=-1}
      mask prompts: OutMin "Simulink:blkprm_prompts:OutputDesignMin"; OutMax "Simulink:blkprm_prompts:OutputDesignMax"; OutDataTypeStr "Simulink:blkprm_prompts:OUTPUT_UNIFIEDDATATYPE"; LockScale "Simulink:blkprm_prompts:LockScale"; ConvertRealWorld "Simulink:blkprm_prompts:DtypeCnvInputOutputValue"; RndMeth "Simulink:blkprm_prompts:SPP_RndMeth_ID"; SaturateOnIntegerOverflow "Simulink:blkprm_prompts:AllBlksSaturate"; SampleTime "Simulink:blkprm_prompts:AllBlksSampleTime"
      mask help:
      | 入力を出力のデータ型とスケーリングに変換します。
      |
      | この変換には 2 つの目的があります。1 つは入力と出力の実際値を等しくすることです。もう 1 つは入力と出力の整数格納値を等しくすることです。オーバーフローと量子化誤差があると、この目的を完全に達成することができません。
      settings: AttributesFormatString=%<Tag>\nOutDataType = %<OutDataTypeStr>
      mask TypeOptions OutMin: OutMin
      mask TypeOptions OutMax: OutMax
      mask TypeOptions OutDataTypeStr: OutDataTypeStr
      mask TypeOptions LockScale: LockScale
      mask TypeOptions ConvertRealWorld: ConvertRealWorld
      mask TypeOptions RndMeth: RndMeth
      mask TypeOptions SaturateOnIntegerOverflow: SaturateOnIntegerOverflow
      mask TypeOptions SampleTime: SampleTime
      mask DialogControl OutMin Prompt: 出力の最小値:
      mask DialogControl OutMax Prompt: 出力の最大値:
      mask DialogControl OutDataTypeStr Prompt: 出力データ型:
      mask DialogControl LockScale Prompt: 固定小数点ツールによる変更に対して出力データ型の設定をロックする
      mask DialogControl ConvertRealWorld Prompt: 等価な値をもつ入力と出力:
      mask DialogControl RndMeth Prompt: 整数丸めモード:
      mask DialogControl SaturateOnIntegerOverflow Prompt: 整数オーバーフローで飽和
      mask DialogControl SampleTime Prompt: サンプル時間 (継承は -1):
  Data Type Conversion6 : DataTypeConversion  Tag=#AMO_Lib  OutMin=OutMin  OutMax=OutMax  OutDataTypeStr=TSB_Tbatt_float  SampleTime=SampleTime  SaturateOnIntegerOverflow=on  RndMeth=Zero  mask{OutMin=[], OutMax=[], OutDataTypeStr=TSB_Tbatt_float, LockScale=off, ConvertRealWorld=Real World Value (RWV), RndMeth=Zero, SaturateOnIntegerOverflow=on, SampleTime=-1}
      mask prompts: OutMin "Simulink:blkprm_prompts:OutputDesignMin"; OutMax "Simulink:blkprm_prompts:OutputDesignMax"; OutDataTypeStr "Simulink:blkprm_prompts:OUTPUT_UNIFIEDDATATYPE"; LockScale "Simulink:blkprm_prompts:LockScale"; ConvertRealWorld "Simulink:blkprm_prompts:DtypeCnvInputOutputValue"; RndMeth "Simulink:blkprm_prompts:SPP_RndMeth_ID"; SaturateOnIntegerOverflow "Simulink:blkprm_prompts:AllBlksSaturate"; SampleTime "Simulink:blkprm_prompts:AllBlksSampleTime"
      mask help:
      | 入力を出力のデータ型とスケーリングに変換します。
      |
      | この変換には 2 つの目的があります。1 つは入力と出力の実際値を等しくすることです。もう 1 つは入力と出力の整数格納値を等しくすることです。オーバーフローと量子化誤差があると、この目的を完全に達成することができません。
      settings: AttributesFormatString=%<Tag>\nOutDataType = %<OutDataTypeStr>
      mask TypeOptions OutMin: OutMin
      mask TypeOptions OutMax: OutMax
      mask TypeOptions OutDataTypeStr: OutDataTypeStr
      mask TypeOptions LockScale: LockScale
      mask TypeOptions ConvertRealWorld: ConvertRealWorld
      mask TypeOptions RndMeth: RndMeth
      mask TypeOptions SaturateOnIntegerOverflow: SaturateOnIntegerOverflow
      mask TypeOptions SampleTime: SampleTime
      mask DialogControl OutMin Prompt: 出力の最小値:
      mask DialogControl OutMax Prompt: 出力の最大値:
      mask DialogControl OutDataTypeStr Prompt: 出力データ型:
      mask DialogControl LockScale Prompt: 固定小数点ツールによる変更に対して出力データ型の設定をロックする
      mask DialogControl ConvertRealWorld Prompt: 等価な値をもつ入力と出力:
      mask DialogControl RndMeth Prompt: 整数丸めモード:
      mask DialogControl SaturateOnIntegerOverflow Prompt: 整数オーバーフローで飽和
      mask DialogControl SampleTime Prompt: サンプル時間 (継承は -1):
  Data Type Conversion7 : DataTypeConversion  Tag=#AMO_Lib  OutMin=OutMin  OutMax=OutMax  OutDataTypeStr=single  ConvertRealWorld=Stored Integer (SI)  SampleTime=SampleTime  SaturateOnIntegerOverflow=on  RndMeth=Zero  mask{OutMin=[], OutMax=[], OutDataTypeStr=single, LockScale=off, ConvertRealWorld=Stored Integer (SI), RndMeth=Zero, SaturateOnIntegerOverflow=on, SampleTime=-1}
      mask prompts: OutMin "Simulink:blkprm_prompts:OutputDesignMin"; OutMax "Simulink:blkprm_prompts:OutputDesignMax"; OutDataTypeStr "Simulink:blkprm_prompts:OUTPUT_UNIFIEDDATATYPE"; LockScale "Simulink:blkprm_prompts:LockScale"; ConvertRealWorld "Simulink:blkprm_prompts:DtypeCnvInputOutputValue"; RndMeth "Simulink:blkprm_prompts:SPP_RndMeth_ID"; SaturateOnIntegerOverflow "Simulink:blkprm_prompts:AllBlksSaturate"; SampleTime "Simulink:blkprm_prompts:AllBlksSampleTime"
      mask help:
      | 入力を出力のデータ型とスケーリングに変換します。
      |
      | この変換には 2 つの目的があります。1 つは入力と出力の実際値を等しくすることです。もう 1 つは入力と出力の整数格納値を等しくすることです。オーバーフローと量子化誤差があると、この目的を完全に達成することができません。
      settings: AttributesFormatString=%<Tag>\nOutDataType = %<OutDataTypeStr>
      mask TypeOptions OutMin: OutMin
      mask TypeOptions OutMax: OutMax
      mask TypeOptions OutDataTypeStr: OutDataTypeStr
      mask TypeOptions LockScale: LockScale
      mask TypeOptions ConvertRealWorld: ConvertRealWorld
      mask TypeOptions RndMeth: RndMeth
      mask TypeOptions SaturateOnIntegerOverflow: SaturateOnIntegerOverflow
      mask TypeOptions SampleTime: SampleTime
      mask DialogControl OutMin Prompt: 出力の最小値:
      mask DialogControl OutMax Prompt: 出力の最大値:
      mask DialogControl OutDataTypeStr Prompt: 出力データ型:
      mask DialogControl LockScale Prompt: 固定小数点ツールによる変更に対して出力データ型の設定をロックする
      mask DialogControl ConvertRealWorld Prompt: 等価な値をもつ入力と出力:
      mask DialogControl RndMeth Prompt: 整数丸めモード:
      mask DialogControl SaturateOnIntegerOverflow Prompt: 整数オーバーフローで飽和
      mask DialogControl SampleTime Prompt: サンプル時間 (継承は -1):
  Data Type Conversion8 : DataTypeConversion  Tag=#AMO_Lib  OutMin=OutMin  OutMax=OutMax  OutDataTypeStr=TSB_Coulomb_float  SampleTime=SampleTime  SaturateOnIntegerOverflow=on  RndMeth=Zero  mask{OutMin=[], OutMax=[], OutDataTypeStr=TSB_Coulomb_float, LockScale=off, ConvertRealWorld=Real World Value (RWV), RndMeth=Zero, SaturateOnIntegerOverflow=on, SampleTime=-1}
      mask prompts: OutMin "Simulink:blkprm_prompts:OutputDesignMin"; OutMax "Simulink:blkprm_prompts:OutputDesignMax"; OutDataTypeStr "Simulink:blkprm_prompts:OUTPUT_UNIFIEDDATATYPE"; LockScale "Simulink:blkprm_prompts:LockScale"; ConvertRealWorld "Simulink:blkprm_prompts:DtypeCnvInputOutputValue"; RndMeth "Simulink:blkprm_prompts:SPP_RndMeth_ID"; SaturateOnIntegerOverflow "Simulink:blkprm_prompts:AllBlksSaturate"; SampleTime "Simulink:blkprm_prompts:AllBlksSampleTime"
      mask help:
      | 入力を出力のデータ型とスケーリングに変換します。
      |
      | この変換には 2 つの目的があります。1 つは入力と出力の実際値を等しくすることです。もう 1 つは入力と出力の整数格納値を等しくすることです。オーバーフローと量子化誤差があると、この目的を完全に達成することができません。
      settings: AttributesFormatString=%<Tag>\nOutDataType = %<OutDataTypeStr>
      mask TypeOptions OutMin: OutMin
      mask TypeOptions OutMax: OutMax
      mask TypeOptions OutDataTypeStr: OutDataTypeStr
      mask TypeOptions LockScale: LockScale
      mask TypeOptions ConvertRealWorld: ConvertRealWorld
      mask TypeOptions RndMeth: RndMeth
      mask TypeOptions SaturateOnIntegerOverflow: SaturateOnIntegerOverflow
      mask TypeOptions SampleTime: SampleTime
      mask DialogControl OutMin Prompt: 出力の最小値:
      mask DialogControl OutMax Prompt: 出力の最大値:
      mask DialogControl OutDataTypeStr Prompt: 出力データ型:
      mask DialogControl LockScale Prompt: 固定小数点ツールによる変更に対して出力データ型の設定をロックする
      mask DialogControl ConvertRealWorld Prompt: 等価な値をもつ入力と出力:
      mask DialogControl RndMeth Prompt: 整数丸めモード:
      mask DialogControl SaturateOnIntegerOverflow Prompt: 整数オーバーフローで飽和
      mask DialogControl SampleTime Prompt: サンプル時間 (継承は -1):
  Data Type Conversion9 : DataTypeConversion  Tag=#AMO_Lib  OutMin=OutMin  OutMax=OutMax  OutDataTypeStr=single  ConvertRealWorld=Stored Integer (SI)  SampleTime=SampleTime  SaturateOnIntegerOverflow=on  RndMeth=Zero  mask{OutMin=[], OutMax=[], OutDataTypeStr=single, LockScale=off, ConvertRealWorld=Stored Integer (SI), RndMeth=Zero, SaturateOnIntegerOverflow=on, SampleTime=-1}
      mask prompts: OutMin "Simulink:blkprm_prompts:OutputDesignMin"; OutMax "Simulink:blkprm_prompts:OutputDesignMax"; OutDataTypeStr "Simulink:blkprm_prompts:OUTPUT_UNIFIEDDATATYPE"; LockScale "Simulink:blkprm_prompts:LockScale"; ConvertRealWorld "Simulink:blkprm_prompts:DtypeCnvInputOutputValue"; RndMeth "Simulink:blkprm_prompts:SPP_RndMeth_ID"; SaturateOnIntegerOverflow "Simulink:blkprm_prompts:AllBlksSaturate"; SampleTime "Simulink:blkprm_prompts:AllBlksSampleTime"
      mask help:
      | 入力を出力のデータ型とスケーリングに変換します。
      |
      | この変換には 2 つの目的があります。1 つは入力と出力の実際値を等しくすることです。もう 1 つは入力と出力の整数格納値を等しくすることです。オーバーフローと量子化誤差があると、この目的を完全に達成することができません。
      settings: AttributesFormatString=%<Tag>\nOutDataType = %<OutDataTypeStr>
      mask TypeOptions OutMin: OutMin
      mask TypeOptions OutMax: OutMax
      mask TypeOptions OutDataTypeStr: OutDataTypeStr
      mask TypeOptions LockScale: LockScale
      mask TypeOptions ConvertRealWorld: ConvertRealWorld
      mask TypeOptions RndMeth: RndMeth
      mask TypeOptions SaturateOnIntegerOverflow: SaturateOnIntegerOverflow
      mask TypeOptions SampleTime: SampleTime
      mask DialogControl OutMin Prompt: 出力の最小値:
      mask DialogControl OutMax Prompt: 出力の最大値:
      mask DialogControl OutDataTypeStr Prompt: 出力データ型:
      mask DialogControl LockScale Prompt: 固定小数点ツールによる変更に対して出力データ型の設定をロックする
      mask DialogControl ConvertRealWorld Prompt: 等価な値をもつ入力と出力:
      mask DialogControl RndMeth Prompt: 整数丸めモード:
      mask DialogControl SaturateOnIntegerOverflow Prompt: 整数オーバーフローで飽和
      mask DialogControl SampleTime Prompt: サンプル時間 (継承は -1):
  Divide : Product  Tag=#AMO_Lib  Inputs=*/  CollapseDim=CollapseDim  OutMin=OutMin  OutMax=OutMax  SampleTime=SampleTime  SaturateOnIntegerOverflow=on  RndMeth=Zero  mask{Inputs=*/, Multiplication=Element-wise(.*), CollapseMode=All dimensions, CollapseDim=1, SampleTime=-1, InputSameDT=off, OutMin=[], OutMax=[], OutDataTypeStr=Inherit: Inherit via internal rule, LockScale=off, RndMeth=Zero, SaturateOnIntegerOverflow=on}
      mask prompts: Inputs "Simulink:blkprm_prompts:ProdNumInputs"; Multiplication "Simulink:blkprm_prompts:ProdMultiplication"; CollapseMode "Simulink:blkprm_prompts:ProdOperationType"; CollapseDim "Simulink:blkprm_prompts:ProdOperationDim"; SampleTime "Simulink:blkprm_prompts:AllBlksSampleTime"; InputSameDT "Simulink:blkprm_prompts:InputSameDT"; OutMin "Simulink:blkprm_prompts:OutputDesignMin"; OutMax "Simulink:blkprm_prompts:OutputDesignMax"; OutDataTypeStr "Simulink:blkprm_prompts:OUTPUT_UNIFIEDDATATYPE"; LockScale "Simulink:blkprm_prompts:LockScale"; RndMeth "Simulink:blkprm_prompts:SPP_RndMeth_ID"; SaturateOnIntegerOverflow "Simulink:blkprm_prompts:AllBlksSaturate"
      mask help:
      | 入力を乗算または除算します。要素単位、または行列の乗算を選択し、以下のいずれかを指定してください:
      |  a) 各入力端子に対して * または /。たとえば、**/* は演算 'u1*u2/u3*u4' を実行します。
      |  b) 乗算を行う入力端子の数を指定するスカラー値。たとえば、2 は演算 'u1*u2' を実行します。
      |
      | 1 つの入力端子のみがあり、乗算パラメーターが要素単位 (.*) に設定されている場合、1 つの * または / は、指定した演算を各要素に適用します。しかし、乗算パラメーターが行列 (*) に設定されている場合、1 つの * は行列の乗算を出力し、1 つの / は逆行列を出力します。
      settings: AttributesFormatString=%<Tag>\nOutDataType = %<OutDataTypeStr>
      mask TypeOptions Inputs: Inputs
      mask TypeOptions Multiplication: Multiplication
      mask TypeOptions CollapseMode: CollapseMode
      mask TypeOptions CollapseDim: CollapseDim
      mask TypeOptions SampleTime: SampleTime
      mask TypeOptions InputSameDT: InputSameDT
      mask TypeOptions OutMin: OutMin
      mask TypeOptions OutMax: OutMax
      mask TypeOptions OutDataTypeStr: OutDataTypeStr
      mask TypeOptions LockScale: LockScale
      mask TypeOptions RndMeth: RndMeth
      mask TypeOptions SaturateOnIntegerOverflow: SaturateOnIntegerOverflow
      mask DialogControl Container7 Prompt: メイン
      mask DialogControl Inputs Prompt: 入力数:
      mask DialogControl Multiplication Prompt: 乗算:
      mask DialogControl CollapseMode Prompt: 乗算範囲:
      mask DialogControl CollapseDim Prompt: 次元:
      mask DialogControl SampleTime Prompt: サンプル時間 (継承は -1):
      mask DialogControl Container8 Prompt: 信号属性
      mask DialogControl InputSameDT Prompt: すべての入力が同じデータ型をもつ
      mask DialogControl OutMin Prompt: 出力の最小値:
      mask DialogControl OutMax Prompt: 出力の最大値:
      mask DialogControl OutDataTypeStr Prompt: 出力データ型:
      mask DialogControl LockScale Prompt: 固定小数点ツールによる変更に対して出力データ型の設定をロックする
      mask DialogControl RndMeth Prompt: 整数丸めモード:
      mask DialogControl SaturateOnIntegerOverflow Prompt: 整数オーバーフローで飽和
  Divide1 : Product  Tag=#AMO_Lib  Inputs=*/  CollapseDim=CollapseDim  OutMin=OutMin  OutMax=OutMax  SampleTime=SampleTime  SaturateOnIntegerOverflow=on  RndMeth=Zero  mask{Inputs=*/, Multiplication=Element-wise(.*), CollapseMode=All dimensions, CollapseDim=1, SampleTime=-1, InputSameDT=off, OutMin=[], OutMax=[], OutDataTypeStr=Inherit: Inherit via internal rule, LockScale=off, RndMeth=Zero, SaturateOnIntegerOverflow=on}
      mask prompts: Inputs "Simulink:blkprm_prompts:ProdNumInputs"; Multiplication "Simulink:blkprm_prompts:ProdMultiplication"; CollapseMode "Simulink:blkprm_prompts:ProdOperationType"; CollapseDim "Simulink:blkprm_prompts:ProdOperationDim"; SampleTime "Simulink:blkprm_prompts:AllBlksSampleTime"; InputSameDT "Simulink:blkprm_prompts:InputSameDT"; OutMin "Simulink:blkprm_prompts:OutputDesignMin"; OutMax "Simulink:blkprm_prompts:OutputDesignMax"; OutDataTypeStr "Simulink:blkprm_prompts:OUTPUT_UNIFIEDDATATYPE"; LockScale "Simulink:blkprm_prompts:LockScale"; RndMeth "Simulink:blkprm_prompts:SPP_RndMeth_ID"; SaturateOnIntegerOverflow "Simulink:blkprm_prompts:AllBlksSaturate"
      mask help:
      | 入力を乗算または除算します。要素単位、または行列の乗算を選択し、以下のいずれかを指定してください:
      |  a) 各入力端子に対して * または /。たとえば、**/* は演算 'u1*u2/u3*u4' を実行します。
      |  b) 乗算を行う入力端子の数を指定するスカラー値。たとえば、2 は演算 'u1*u2' を実行します。
      |
      | 1 つの入力端子のみがあり、乗算パラメーターが要素単位 (.*) に設定されている場合、1 つの * または / は、指定した演算を各要素に適用します。しかし、乗算パラメーターが行列 (*) に設定されている場合、1 つの * は行列の乗算を出力し、1 つの / は逆行列を出力します。
      settings: AttributesFormatString=%<Tag>\nOutDataType = %<OutDataTypeStr>
      mask TypeOptions Inputs: Inputs
      mask TypeOptions Multiplication: Multiplication
      mask TypeOptions CollapseMode: CollapseMode
      mask TypeOptions CollapseDim: CollapseDim
      mask TypeOptions SampleTime: SampleTime
      mask TypeOptions InputSameDT: InputSameDT
      mask TypeOptions OutMin: OutMin
      mask TypeOptions OutMax: OutMax
      mask TypeOptions OutDataTypeStr: OutDataTypeStr
      mask TypeOptions LockScale: LockScale
      mask TypeOptions RndMeth: RndMeth
      mask TypeOptions SaturateOnIntegerOverflow: SaturateOnIntegerOverflow
      mask DialogControl Container7 Prompt: メイン
      mask DialogControl Inputs Prompt: 入力数:
      mask DialogControl Multiplication Prompt: 乗算:
      mask DialogControl CollapseMode Prompt: 乗算範囲:
      mask DialogControl CollapseDim Prompt: 次元:
      mask DialogControl SampleTime Prompt: サンプル時間 (継承は -1):
      mask DialogControl Container8 Prompt: 信号属性
      mask DialogControl InputSameDT Prompt: すべての入力が同じデータ型をもつ
      mask DialogControl OutMin Prompt: 出力の最小値:
      mask DialogControl OutMax Prompt: 出力の最大値:
      mask DialogControl OutDataTypeStr Prompt: 出力データ型:
      mask DialogControl LockScale Prompt: 固定小数点ツールによる変更に対して出力データ型の設定をロックする
      mask DialogControl RndMeth Prompt: 整数丸めモード:
      mask DialogControl SaturateOnIntegerOverflow Prompt: 整数オーバーフローで飽和
  Divide10 : Product  Tag=#AMO_Lib  Inputs=*/  CollapseDim=CollapseDim  OutMin=OutMin  OutMax=OutMax  SampleTime=SampleTime  SaturateOnIntegerOverflow=on  RndMeth=Zero  mask{Inputs=*/, Multiplication=Element-wise(.*), CollapseMode=All dimensions, CollapseDim=1, SampleTime=-1, InputSameDT=off, OutMin=[], OutMax=[], OutDataTypeStr=Inherit: Inherit via internal rule, LockScale=off, RndMeth=Zero, SaturateOnIntegerOverflow=on}
      mask prompts: Inputs "Simulink:blkprm_prompts:ProdNumInputs"; Multiplication "Simulink:blkprm_prompts:ProdMultiplication"; CollapseMode "Simulink:blkprm_prompts:ProdOperationType"; CollapseDim "Simulink:blkprm_prompts:ProdOperationDim"; SampleTime "Simulink:blkprm_prompts:AllBlksSampleTime"; InputSameDT "Simulink:blkprm_prompts:InputSameDT"; OutMin "Simulink:blkprm_prompts:OutputDesignMin"; OutMax "Simulink:blkprm_prompts:OutputDesignMax"; OutDataTypeStr "Simulink:blkprm_prompts:OUTPUT_UNIFIEDDATATYPE"; LockScale "Simulink:blkprm_prompts:LockScale"; RndMeth "Simulink:blkprm_prompts:SPP_RndMeth_ID"; SaturateOnIntegerOverflow "Simulink:blkprm_prompts:AllBlksSaturate"
      mask help:
      | 入力を乗算または除算します。要素単位、または行列の乗算を選択し、以下のいずれかを指定してください:
      |  a) 各入力端子に対して * または /。たとえば、**/* は演算 'u1*u2/u3*u4' を実行します。
      |  b) 乗算を行う入力端子の数を指定するスカラー値。たとえば、2 は演算 'u1*u2' を実行します。
      |
      | 1 つの入力端子のみがあり、乗算パラメーターが要素単位 (.*) に設定されている場合、1 つの * または / は、指定した演算を各要素に適用します。しかし、乗算パラメーターが行列 (*) に設定されている場合、1 つの * は行列の乗算を出力し、1 つの / は逆行列を出力します。
      settings: AttributesFormatString=%<Tag>\nOutDataType = %<OutDataTypeStr>
      mask TypeOptions Inputs: Inputs
      mask TypeOptions Multiplication: Multiplication
      mask TypeOptions CollapseMode: CollapseMode
      mask TypeOptions CollapseDim: CollapseDim
      mask TypeOptions SampleTime: SampleTime
      mask TypeOptions InputSameDT: InputSameDT
      mask TypeOptions OutMin: OutMin
      mask TypeOptions OutMax: OutMax
      mask TypeOptions OutDataTypeStr: OutDataTypeStr
      mask TypeOptions LockScale: LockScale
      mask TypeOptions RndMeth: RndMeth
      mask TypeOptions SaturateOnIntegerOverflow: SaturateOnIntegerOverflow
      mask DialogControl Container7 Prompt: メイン
      mask DialogControl Inputs Prompt: 入力数:
      mask DialogControl Multiplication Prompt: 乗算:
      mask DialogControl CollapseMode Prompt: 乗算範囲:
      mask DialogControl CollapseDim Prompt: 次元:
      mask DialogControl SampleTime Prompt: サンプル時間 (継承は -1):
      mask DialogControl Container8 Prompt: 信号属性
      mask DialogControl InputSameDT Prompt: すべての入力が同じデータ型をもつ
      mask DialogControl OutMin Prompt: 出力の最小値:
      mask DialogControl OutMax Prompt: 出力の最大値:
      mask DialogControl OutDataTypeStr Prompt: 出力データ型:
      mask DialogControl LockScale Prompt: 固定小数点ツールによる変更に対して出力データ型の設定をロックする
      mask DialogControl RndMeth Prompt: 整数丸めモード:
      mask DialogControl SaturateOnIntegerOverflow Prompt: 整数オーバーフローで飽和
  Divide2 : Product  Tag=#AMO_Lib  Inputs=*/  CollapseDim=CollapseDim  OutMin=OutMin  OutMax=OutMax  SampleTime=SampleTime  SaturateOnIntegerOverflow=on  RndMeth=Zero  mask{Inputs=*/, Multiplication=Element-wise(.*), CollapseMode=All dimensions, CollapseDim=1, SampleTime=-1, InputSameDT=off, OutMin=[], OutMax=[], OutDataTypeStr=Inherit: Inherit via internal rule, LockScale=off, RndMeth=Zero, SaturateOnIntegerOverflow=on}
      mask prompts: Inputs "Simulink:blkprm_prompts:ProdNumInputs"; Multiplication "Simulink:blkprm_prompts:ProdMultiplication"; CollapseMode "Simulink:blkprm_prompts:ProdOperationType"; CollapseDim "Simulink:blkprm_prompts:ProdOperationDim"; SampleTime "Simulink:blkprm_prompts:AllBlksSampleTime"; InputSameDT "Simulink:blkprm_prompts:InputSameDT"; OutMin "Simulink:blkprm_prompts:OutputDesignMin"; OutMax "Simulink:blkprm_prompts:OutputDesignMax"; OutDataTypeStr "Simulink:blkprm_prompts:OUTPUT_UNIFIEDDATATYPE"; LockScale "Simulink:blkprm_prompts:LockScale"; RndMeth "Simulink:blkprm_prompts:SPP_RndMeth_ID"; SaturateOnIntegerOverflow "Simulink:blkprm_prompts:AllBlksSaturate"
      mask help:
      | 入力を乗算または除算します。要素単位、または行列の乗算を選択し、以下のいずれかを指定してください:
      |  a) 各入力端子に対して * または /。たとえば、**/* は演算 'u1*u2/u3*u4' を実行します。
      |  b) 乗算を行う入力端子の数を指定するスカラー値。たとえば、2 は演算 'u1*u2' を実行します。
      |
      | 1 つの入力端子のみがあり、乗算パラメーターが要素単位 (.*) に設定されている場合、1 つの * または / は、指定した演算を各要素に適用します。しかし、乗算パラメーターが行列 (*) に設定されている場合、1 つの * は行列の乗算を出力し、1 つの / は逆行列を出力します。
      settings: AttributesFormatString=%<Tag>\nOutDataType = %<OutDataTypeStr>
      mask TypeOptions Inputs: Inputs
      mask TypeOptions Multiplication: Multiplication
      mask TypeOptions CollapseMode: CollapseMode
      mask TypeOptions CollapseDim: CollapseDim
      mask TypeOptions SampleTime: SampleTime
      mask TypeOptions InputSameDT: InputSameDT
      mask TypeOptions OutMin: OutMin
      mask TypeOptions OutMax: OutMax
      mask TypeOptions OutDataTypeStr: OutDataTypeStr
      mask TypeOptions LockScale: LockScale
      mask TypeOptions RndMeth: RndMeth
      mask TypeOptions SaturateOnIntegerOverflow: SaturateOnIntegerOverflow
      mask DialogControl Container7 Prompt: メイン
      mask DialogControl Inputs Prompt: 入力数:
      mask DialogControl Multiplication Prompt: 乗算:
      mask DialogControl CollapseMode Prompt: 乗算範囲:
      mask DialogControl CollapseDim Prompt: 次元:
      mask DialogControl SampleTime Prompt: サンプル時間 (継承は -1):
      mask DialogControl Container8 Prompt: 信号属性
      mask DialogControl InputSameDT Prompt: すべての入力が同じデータ型をもつ
      mask DialogControl OutMin Prompt: 出力の最小値:
      mask DialogControl OutMax Prompt: 出力の最大値:
      mask DialogControl OutDataTypeStr Prompt: 出力データ型:
      mask DialogControl LockScale Prompt: 固定小数点ツールによる変更に対して出力データ型の設定をロックする
      mask DialogControl RndMeth Prompt: 整数丸めモード:
      mask DialogControl SaturateOnIntegerOverflow Prompt: 整数オーバーフローで飽和
  Divide3 : Product  Tag=#AMO_Lib  Inputs=*/  CollapseDim=CollapseDim  OutMin=OutMin  OutMax=OutMax  SampleTime=SampleTime  SaturateOnIntegerOverflow=on  RndMeth=Zero  mask{Inputs=*/, Multiplication=Element-wise(.*), CollapseMode=All dimensions, CollapseDim=1, SampleTime=-1, InputSameDT=off, OutMin=[], OutMax=[], OutDataTypeStr=Inherit: Inherit via internal rule, LockScale=off, RndMeth=Zero, SaturateOnIntegerOverflow=on}
      mask prompts: Inputs "Simulink:blkprm_prompts:ProdNumInputs"; Multiplication "Simulink:blkprm_prompts:ProdMultiplication"; CollapseMode "Simulink:blkprm_prompts:ProdOperationType"; CollapseDim "Simulink:blkprm_prompts:ProdOperationDim"; SampleTime "Simulink:blkprm_prompts:AllBlksSampleTime"; InputSameDT "Simulink:blkprm_prompts:InputSameDT"; OutMin "Simulink:blkprm_prompts:OutputDesignMin"; OutMax "Simulink:blkprm_prompts:OutputDesignMax"; OutDataTypeStr "Simulink:blkprm_prompts:OUTPUT_UNIFIEDDATATYPE"; LockScale "Simulink:blkprm_prompts:LockScale"; RndMeth "Simulink:blkprm_prompts:SPP_RndMeth_ID"; SaturateOnIntegerOverflow "Simulink:blkprm_prompts:AllBlksSaturate"
      mask help:
      | 入力を乗算または除算します。要素単位、または行列の乗算を選択し、以下のいずれかを指定してください:
      |  a) 各入力端子に対して * または /。たとえば、**/* は演算 'u1*u2/u3*u4' を実行します。
      |  b) 乗算を行う入力端子の数を指定するスカラー値。たとえば、2 は演算 'u1*u2' を実行します。
      |
      | 1 つの入力端子のみがあり、乗算パラメーターが要素単位 (.*) に設定されている場合、1 つの * または / は、指定した演算を各要素に適用します。しかし、乗算パラメーターが行列 (*) に設定されている場合、1 つの * は行列の乗算を出力し、1 つの / は逆行列を出力します。
      settings: AttributesFormatString=%<Tag>\nOutDataType = %<OutDataTypeStr>
      mask TypeOptions Inputs: Inputs
      mask TypeOptions Multiplication: Multiplication
      mask TypeOptions CollapseMode: CollapseMode
      mask TypeOptions CollapseDim: CollapseDim
      mask TypeOptions SampleTime: SampleTime
      mask TypeOptions InputSameDT: InputSameDT
      mask TypeOptions OutMin: OutMin
      mask TypeOptions OutMax: OutMax
      mask TypeOptions OutDataTypeStr: OutDataTypeStr
      mask TypeOptions LockScale: LockScale
      mask TypeOptions RndMeth: RndMeth
      mask TypeOptions SaturateOnIntegerOverflow: SaturateOnIntegerOverflow
      mask DialogControl Container7 Prompt: メイン
      mask DialogControl Inputs Prompt: 入力数:
      mask DialogControl Multiplication Prompt: 乗算:
      mask DialogControl CollapseMode Prompt: 乗算範囲:
      mask DialogControl CollapseDim Prompt: 次元:
      mask DialogControl SampleTime Prompt: サンプル時間 (継承は -1):
      mask DialogControl Container8 Prompt: 信号属性
      mask DialogControl InputSameDT Prompt: すべての入力が同じデータ型をもつ
      mask DialogControl OutMin Prompt: 出力の最小値:
      mask DialogControl OutMax Prompt: 出力の最大値:
      mask DialogControl OutDataTypeStr Prompt: 出力データ型:
      mask DialogControl LockScale Prompt: 固定小数点ツールによる変更に対して出力データ型の設定をロックする
      mask DialogControl RndMeth Prompt: 整数丸めモード:
      mask DialogControl SaturateOnIntegerOverflow Prompt: 整数オーバーフローで飽和
  Divide4 : Product  Tag=#AMO_Lib  Inputs=*/  CollapseDim=CollapseDim  OutMin=OutMin  OutMax=OutMax  SampleTime=SampleTime  SaturateOnIntegerOverflow=on  RndMeth=Zero  mask{Inputs=*/, Multiplication=Element-wise(.*), CollapseMode=All dimensions, CollapseDim=1, SampleTime=-1, InputSameDT=off, OutMin=[], OutMax=[], OutDataTypeStr=Inherit: Inherit via internal rule, LockScale=off, RndMeth=Zero, SaturateOnIntegerOverflow=on}
      mask prompts: Inputs "Simulink:blkprm_prompts:ProdNumInputs"; Multiplication "Simulink:blkprm_prompts:ProdMultiplication"; CollapseMode "Simulink:blkprm_prompts:ProdOperationType"; CollapseDim "Simulink:blkprm_prompts:ProdOperationDim"; SampleTime "Simulink:blkprm_prompts:AllBlksSampleTime"; InputSameDT "Simulink:blkprm_prompts:InputSameDT"; OutMin "Simulink:blkprm_prompts:OutputDesignMin"; OutMax "Simulink:blkprm_prompts:OutputDesignMax"; OutDataTypeStr "Simulink:blkprm_prompts:OUTPUT_UNIFIEDDATATYPE"; LockScale "Simulink:blkprm_prompts:LockScale"; RndMeth "Simulink:blkprm_prompts:SPP_RndMeth_ID"; SaturateOnIntegerOverflow "Simulink:blkprm_prompts:AllBlksSaturate"
      mask help:
      | 入力を乗算または除算します。要素単位、または行列の乗算を選択し、以下のいずれかを指定してください:
      |  a) 各入力端子に対して * または /。たとえば、**/* は演算 'u1*u2/u3*u4' を実行します。
      |  b) 乗算を行う入力端子の数を指定するスカラー値。たとえば、2 は演算 'u1*u2' を実行します。
      |
      | 1 つの入力端子のみがあり、乗算パラメーターが要素単位 (.*) に設定されている場合、1 つの * または / は、指定した演算を各要素に適用します。しかし、乗算パラメーターが行列 (*) に設定されている場合、1 つの * は行列の乗算を出力し、1 つの / は逆行列を出力します。
      settings: AttributesFormatString=%<Tag>\nOutDataType = %<OutDataTypeStr>
      mask TypeOptions Inputs: Inputs
      mask TypeOptions Multiplication: Multiplication
      mask TypeOptions CollapseMode: CollapseMode
      mask TypeOptions CollapseDim: CollapseDim
      mask TypeOptions SampleTime: SampleTime
      mask TypeOptions InputSameDT: InputSameDT
      mask TypeOptions OutMin: OutMin
      mask TypeOptions OutMax: OutMax
      mask TypeOptions OutDataTypeStr: OutDataTypeStr
      mask TypeOptions LockScale: LockScale
      mask TypeOptions RndMeth: RndMeth
      mask TypeOptions SaturateOnIntegerOverflow: SaturateOnIntegerOverflow
      mask DialogControl Container7 Prompt: メイン
      mask DialogControl Inputs Prompt: 入力数:
      mask DialogControl Multiplication Prompt: 乗算:
      mask DialogControl CollapseMode Prompt: 乗算範囲:
      mask DialogControl CollapseDim Prompt: 次元:
      mask DialogControl SampleTime Prompt: サンプル時間 (継承は -1):
      mask DialogControl Container8 Prompt: 信号属性
      mask DialogControl InputSameDT Prompt: すべての入力が同じデータ型をもつ
      mask DialogControl OutMin Prompt: 出力の最小値:
      mask DialogControl OutMax Prompt: 出力の最大値:
      mask DialogControl OutDataTypeStr Prompt: 出力データ型:
      mask DialogControl LockScale Prompt: 固定小数点ツールによる変更に対して出力データ型の設定をロックする
      mask DialogControl RndMeth Prompt: 整数丸めモード:
      mask DialogControl SaturateOnIntegerOverflow Prompt: 整数オーバーフローで飽和
  Divide5 : Product  Tag=#AMO_Lib  Inputs=*/  CollapseDim=CollapseDim  OutMin=OutMin  OutMax=OutMax  SampleTime=SampleTime  SaturateOnIntegerOverflow=on  RndMeth=Zero  mask{Inputs=*/, Multiplication=Element-wise(.*), CollapseMode=All dimensions, CollapseDim=1, SampleTime=-1, InputSameDT=off, OutMin=[], OutMax=[], OutDataTypeStr=Inherit: Inherit via internal rule, LockScale=off, RndMeth=Zero, SaturateOnIntegerOverflow=on}
      mask prompts: Inputs "Simulink:blkprm_prompts:ProdNumInputs"; Multiplication "Simulink:blkprm_prompts:ProdMultiplication"; CollapseMode "Simulink:blkprm_prompts:ProdOperationType"; CollapseDim "Simulink:blkprm_prompts:ProdOperationDim"; SampleTime "Simulink:blkprm_prompts:AllBlksSampleTime"; InputSameDT "Simulink:blkprm_prompts:InputSameDT"; OutMin "Simulink:blkprm_prompts:OutputDesignMin"; OutMax "Simulink:blkprm_prompts:OutputDesignMax"; OutDataTypeStr "Simulink:blkprm_prompts:OUTPUT_UNIFIEDDATATYPE"; LockScale "Simulink:blkprm_prompts:LockScale"; RndMeth "Simulink:blkprm_prompts:SPP_RndMeth_ID"; SaturateOnIntegerOverflow "Simulink:blkprm_prompts:AllBlksSaturate"
      mask help:
      | 入力を乗算または除算します。要素単位、または行列の乗算を選択し、以下のいずれかを指定してください:
      |  a) 各入力端子に対して * または /。たとえば、**/* は演算 'u1*u2/u3*u4' を実行します。
      |  b) 乗算を行う入力端子の数を指定するスカラー値。たとえば、2 は演算 'u1*u2' を実行します。
      |
      | 1 つの入力端子のみがあり、乗算パラメーターが要素単位 (.*) に設定されている場合、1 つの * または / は、指定した演算を各要素に適用します。しかし、乗算パラメーターが行列 (*) に設定されている場合、1 つの * は行列の乗算を出力し、1 つの / は逆行列を出力します。
      settings: AttributesFormatString=%<Tag>\nOutDataType = %<OutDataTypeStr>
      mask TypeOptions Inputs: Inputs
      mask TypeOptions Multiplication: Multiplication
      mask TypeOptions CollapseMode: CollapseMode
      mask TypeOptions CollapseDim: CollapseDim
      mask TypeOptions SampleTime: SampleTime
      mask TypeOptions InputSameDT: InputSameDT
      mask TypeOptions OutMin: OutMin
      mask TypeOptions OutMax: OutMax
      mask TypeOptions OutDataTypeStr: OutDataTypeStr
      mask TypeOptions LockScale: LockScale
      mask TypeOptions RndMeth: RndMeth
      mask TypeOptions SaturateOnIntegerOverflow: SaturateOnIntegerOverflow
      mask DialogControl Container7 Prompt: メイン
      mask DialogControl Inputs Prompt: 入力数:
      mask DialogControl Multiplication Prompt: 乗算:
      mask DialogControl CollapseMode Prompt: 乗算範囲:
      mask DialogControl CollapseDim Prompt: 次元:
      mask DialogControl SampleTime Prompt: サンプル時間 (継承は -1):
      mask DialogControl Container8 Prompt: 信号属性
      mask DialogControl InputSameDT Prompt: すべての入力が同じデータ型をもつ
      mask DialogControl OutMin Prompt: 出力の最小値:
      mask DialogControl OutMax Prompt: 出力の最大値:
      mask DialogControl OutDataTypeStr Prompt: 出力データ型:
      mask DialogControl LockScale Prompt: 固定小数点ツールによる変更に対して出力データ型の設定をロックする
      mask DialogControl RndMeth Prompt: 整数丸めモード:
      mask DialogControl SaturateOnIntegerOverflow Prompt: 整数オーバーフローで飽和
  Divide6 : Product  Tag=#AMO_Lib  Inputs=*/  CollapseDim=CollapseDim  OutMin=OutMin  OutMax=OutMax  SampleTime=SampleTime  SaturateOnIntegerOverflow=on  RndMeth=Zero  mask{Inputs=*/, Multiplication=Element-wise(.*), CollapseMode=All dimensions, CollapseDim=1, SampleTime=-1, InputSameDT=off, OutMin=[], OutMax=[], OutDataTypeStr=Inherit: Inherit via internal rule, LockScale=off, RndMeth=Zero, SaturateOnIntegerOverflow=on}
      mask prompts: Inputs "Simulink:blkprm_prompts:ProdNumInputs"; Multiplication "Simulink:blkprm_prompts:ProdMultiplication"; CollapseMode "Simulink:blkprm_prompts:ProdOperationType"; CollapseDim "Simulink:blkprm_prompts:ProdOperationDim"; SampleTime "Simulink:blkprm_prompts:AllBlksSampleTime"; InputSameDT "Simulink:blkprm_prompts:InputSameDT"; OutMin "Simulink:blkprm_prompts:OutputDesignMin"; OutMax "Simulink:blkprm_prompts:OutputDesignMax"; OutDataTypeStr "Simulink:blkprm_prompts:OUTPUT_UNIFIEDDATATYPE"; LockScale "Simulink:blkprm_prompts:LockScale"; RndMeth "Simulink:blkprm_prompts:SPP_RndMeth_ID"; SaturateOnIntegerOverflow "Simulink:blkprm_prompts:AllBlksSaturate"
      mask help:
      | 入力を乗算または除算します。要素単位、または行列の乗算を選択し、以下のいずれかを指定してください:
      |  a) 各入力端子に対して * または /。たとえば、**/* は演算 'u1*u2/u3*u4' を実行します。
      |  b) 乗算を行う入力端子の数を指定するスカラー値。たとえば、2 は演算 'u1*u2' を実行します。
      |
      | 1 つの入力端子のみがあり、乗算パラメーターが要素単位 (.*) に設定されている場合、1 つの * または / は、指定した演算を各要素に適用します。しかし、乗算パラメーターが行列 (*) に設定されている場合、1 つの * は行列の乗算を出力し、1 つの / は逆行列を出力します。
      settings: AttributesFormatString=%<Tag>\nOutDataType = %<OutDataTypeStr>
      mask TypeOptions Inputs: Inputs
      mask TypeOptions Multiplication: Multiplication
      mask TypeOptions CollapseMode: CollapseMode
      mask TypeOptions CollapseDim: CollapseDim
      mask TypeOptions SampleTime: SampleTime
      mask TypeOptions InputSameDT: InputSameDT
      mask TypeOptions OutMin: OutMin
      mask TypeOptions OutMax: OutMax
      mask TypeOptions OutDataTypeStr: OutDataTypeStr
      mask TypeOptions LockScale: LockScale
      mask TypeOptions RndMeth: RndMeth
      mask TypeOptions SaturateOnIntegerOverflow: SaturateOnIntegerOverflow
      mask DialogControl Container7 Prompt: メイン
      mask DialogControl Inputs Prompt: 入力数:
      mask DialogControl Multiplication Prompt: 乗算:
      mask DialogControl CollapseMode Prompt: 乗算範囲:
      mask DialogControl CollapseDim Prompt: 次元:
      mask DialogControl SampleTime Prompt: サンプル時間 (継承は -1):
      mask DialogControl Container8 Prompt: 信号属性
      mask DialogControl InputSameDT Prompt: すべての入力が同じデータ型をもつ
      mask DialogControl OutMin Prompt: 出力の最小値:
      mask DialogControl OutMax Prompt: 出力の最大値:
      mask DialogControl OutDataTypeStr Prompt: 出力データ型:
      mask DialogControl LockScale Prompt: 固定小数点ツールによる変更に対して出力データ型の設定をロックする
      mask DialogControl RndMeth Prompt: 整数丸めモード:
      mask DialogControl SaturateOnIntegerOverflow Prompt: 整数オーバーフローで飽和
  Divide7 : Product  Tag=#AMO_Lib  Inputs=*/  CollapseDim=CollapseDim  OutMin=OutMin  OutMax=OutMax  SampleTime=SampleTime  SaturateOnIntegerOverflow=on  RndMeth=Zero  mask{Inputs=*/, Multiplication=Element-wise(.*), CollapseMode=All dimensions, CollapseDim=1, SampleTime=-1, InputSameDT=off, OutMin=[], OutMax=[], OutDataTypeStr=Inherit: Inherit via internal rule, LockScale=off, RndMeth=Zero, SaturateOnIntegerOverflow=on}
      mask prompts: Inputs "Simulink:blkprm_prompts:ProdNumInputs"; Multiplication "Simulink:blkprm_prompts:ProdMultiplication"; CollapseMode "Simulink:blkprm_prompts:ProdOperationType"; CollapseDim "Simulink:blkprm_prompts:ProdOperationDim"; SampleTime "Simulink:blkprm_prompts:AllBlksSampleTime"; InputSameDT "Simulink:blkprm_prompts:InputSameDT"; OutMin "Simulink:blkprm_prompts:OutputDesignMin"; OutMax "Simulink:blkprm_prompts:OutputDesignMax"; OutDataTypeStr "Simulink:blkprm_prompts:OUTPUT_UNIFIEDDATATYPE"; LockScale "Simulink:blkprm_prompts:LockScale"; RndMeth "Simulink:blkprm_prompts:SPP_RndMeth_ID"; SaturateOnIntegerOverflow "Simulink:blkprm_prompts:AllBlksSaturate"
      mask help:
      | 入力を乗算または除算します。要素単位、または行列の乗算を選択し、以下のいずれかを指定してください:
      |  a) 各入力端子に対して * または /。たとえば、**/* は演算 'u1*u2/u3*u4' を実行します。
      |  b) 乗算を行う入力端子の数を指定するスカラー値。たとえば、2 は演算 'u1*u2' を実行します。
      |
      | 1 つの入力端子のみがあり、乗算パラメーターが要素単位 (.*) に設定されている場合、1 つの * または / は、指定した演算を各要素に適用します。しかし、乗算パラメーターが行列 (*) に設定されている場合、1 つの * は行列の乗算を出力し、1 つの / は逆行列を出力します。
      settings: AttributesFormatString=%<Tag>\nOutDataType = %<OutDataTypeStr>
      mask TypeOptions Inputs: Inputs
      mask TypeOptions Multiplication: Multiplication
      mask TypeOptions CollapseMode: CollapseMode
      mask TypeOptions CollapseDim: CollapseDim
      mask TypeOptions SampleTime: SampleTime
      mask TypeOptions InputSameDT: InputSameDT
      mask TypeOptions OutMin: OutMin
      mask TypeOptions OutMax: OutMax
      mask TypeOptions OutDataTypeStr: OutDataTypeStr
      mask TypeOptions LockScale: LockScale
      mask TypeOptions RndMeth: RndMeth
      mask TypeOptions SaturateOnIntegerOverflow: SaturateOnIntegerOverflow
      mask DialogControl Container7 Prompt: メイン
      mask DialogControl Inputs Prompt: 入力数:
      mask DialogControl Multiplication Prompt: 乗算:
      mask DialogControl CollapseMode Prompt: 乗算範囲:
      mask DialogControl CollapseDim Prompt: 次元:
      mask DialogControl SampleTime Prompt: サンプル時間 (継承は -1):
      mask DialogControl Container8 Prompt: 信号属性
      mask DialogControl InputSameDT Prompt: すべての入力が同じデータ型をもつ
      mask DialogControl OutMin Prompt: 出力の最小値:
      mask DialogControl OutMax Prompt: 出力の最大値:
      mask DialogControl OutDataTypeStr Prompt: 出力データ型:
      mask DialogControl LockScale Prompt: 固定小数点ツールによる変更に対して出力データ型の設定をロックする
      mask DialogControl RndMeth Prompt: 整数丸めモード:
      mask DialogControl SaturateOnIntegerOverflow Prompt: 整数オーバーフローで飽和
  Divide8 : Product  Tag=#AMO_Lib  Inputs=*/  CollapseDim=CollapseDim  OutMin=OutMin  OutMax=OutMax  SampleTime=SampleTime  SaturateOnIntegerOverflow=on  RndMeth=Zero  mask{Inputs=*/, Multiplication=Element-wise(.*), CollapseMode=All dimensions, CollapseDim=1, SampleTime=-1, InputSameDT=off, OutMin=[], OutMax=[], OutDataTypeStr=Inherit: Inherit via internal rule, LockScale=off, RndMeth=Zero, SaturateOnIntegerOverflow=on}
      mask prompts: Inputs "Simulink:blkprm_prompts:ProdNumInputs"; Multiplication "Simulink:blkprm_prompts:ProdMultiplication"; CollapseMode "Simulink:blkprm_prompts:ProdOperationType"; CollapseDim "Simulink:blkprm_prompts:ProdOperationDim"; SampleTime "Simulink:blkprm_prompts:AllBlksSampleTime"; InputSameDT "Simulink:blkprm_prompts:InputSameDT"; OutMin "Simulink:blkprm_prompts:OutputDesignMin"; OutMax "Simulink:blkprm_prompts:OutputDesignMax"; OutDataTypeStr "Simulink:blkprm_prompts:OUTPUT_UNIFIEDDATATYPE"; LockScale "Simulink:blkprm_prompts:LockScale"; RndMeth "Simulink:blkprm_prompts:SPP_RndMeth_ID"; SaturateOnIntegerOverflow "Simulink:blkprm_prompts:AllBlksSaturate"
      mask help:
      | 入力を乗算または除算します。要素単位、または行列の乗算を選択し、以下のいずれかを指定してください:
      |  a) 各入力端子に対して * または /。たとえば、**/* は演算 'u1*u2/u3*u4' を実行します。
      |  b) 乗算を行う入力端子の数を指定するスカラー値。たとえば、2 は演算 'u1*u2' を実行します。
      |
      | 1 つの入力端子のみがあり、乗算パラメーターが要素単位 (.*) に設定されている場合、1 つの * または / は、指定した演算を各要素に適用します。しかし、乗算パラメーターが行列 (*) に設定されている場合、1 つの * は行列の乗算を出力し、1 つの / は逆行列を出力します。
      settings: AttributesFormatString=%<Tag>\nOutDataType = %<OutDataTypeStr>
      mask TypeOptions Inputs: Inputs
      mask TypeOptions Multiplication: Multiplication
      mask TypeOptions CollapseMode: CollapseMode
      mask TypeOptions CollapseDim: CollapseDim
      mask TypeOptions SampleTime: SampleTime
      mask TypeOptions InputSameDT: InputSameDT
      mask TypeOptions OutMin: OutMin
      mask TypeOptions OutMax: OutMax
      mask TypeOptions OutDataTypeStr: OutDataTypeStr
      mask TypeOptions LockScale: LockScale
      mask TypeOptions RndMeth: RndMeth
      mask TypeOptions SaturateOnIntegerOverflow: SaturateOnIntegerOverflow
      mask DialogControl Container7 Prompt: メイン
      mask DialogControl Inputs Prompt: 入力数:
      mask DialogControl Multiplication Prompt: 乗算:
      mask DialogControl CollapseMode Prompt: 乗算範囲:
      mask DialogControl CollapseDim Prompt: 次元:
      mask DialogControl SampleTime Prompt: サンプル時間 (継承は -1):
      mask DialogControl Container8 Prompt: 信号属性
      mask DialogControl InputSameDT Prompt: すべての入力が同じデータ型をもつ
      mask DialogControl OutMin Prompt: 出力の最小値:
      mask DialogControl OutMax Prompt: 出力の最大値:
      mask DialogControl OutDataTypeStr Prompt: 出力データ型:
      mask DialogControl LockScale Prompt: 固定小数点ツールによる変更に対して出力データ型の設定をロックする
      mask DialogControl RndMeth Prompt: 整数丸めモード:
      mask DialogControl SaturateOnIntegerOverflow Prompt: 整数オーバーフローで飽和
  Divide9 : Product  Tag=#AMO_Lib  Inputs=*/  CollapseDim=CollapseDim  OutMin=OutMin  OutMax=OutMax  SampleTime=SampleTime  SaturateOnIntegerOverflow=on  RndMeth=Zero  mask{Inputs=*/, Multiplication=Element-wise(.*), CollapseMode=All dimensions, CollapseDim=1, SampleTime=-1, InputSameDT=off, OutMin=[], OutMax=[], OutDataTypeStr=Inherit: Inherit via internal rule, LockScale=off, RndMeth=Zero, SaturateOnIntegerOverflow=on}
      mask prompts: Inputs "Simulink:blkprm_prompts:ProdNumInputs"; Multiplication "Simulink:blkprm_prompts:ProdMultiplication"; CollapseMode "Simulink:blkprm_prompts:ProdOperationType"; CollapseDim "Simulink:blkprm_prompts:ProdOperationDim"; SampleTime "Simulink:blkprm_prompts:AllBlksSampleTime"; InputSameDT "Simulink:blkprm_prompts:InputSameDT"; OutMin "Simulink:blkprm_prompts:OutputDesignMin"; OutMax "Simulink:blkprm_prompts:OutputDesignMax"; OutDataTypeStr "Simulink:blkprm_prompts:OUTPUT_UNIFIEDDATATYPE"; LockScale "Simulink:blkprm_prompts:LockScale"; RndMeth "Simulink:blkprm_prompts:SPP_RndMeth_ID"; SaturateOnIntegerOverflow "Simulink:blkprm_prompts:AllBlksSaturate"
      mask help:
      | 入力を乗算または除算します。要素単位、または行列の乗算を選択し、以下のいずれかを指定してください:
      |  a) 各入力端子に対して * または /。たとえば、**/* は演算 'u1*u2/u3*u4' を実行します。
      |  b) 乗算を行う入力端子の数を指定するスカラー値。たとえば、2 は演算 'u1*u2' を実行します。
      |
      | 1 つの入力端子のみがあり、乗算パラメーターが要素単位 (.*) に設定されている場合、1 つの * または / は、指定した演算を各要素に適用します。しかし、乗算パラメーターが行列 (*) に設定されている場合、1 つの * は行列の乗算を出力し、1 つの / は逆行列を出力します。
      settings: AttributesFormatString=%<Tag>\nOutDataType = %<OutDataTypeStr>
      mask TypeOptions Inputs: Inputs
      mask TypeOptions Multiplication: Multiplication
      mask TypeOptions CollapseMode: CollapseMode
      mask TypeOptions CollapseDim: CollapseDim
      mask TypeOptions SampleTime: SampleTime
      mask TypeOptions InputSameDT: InputSameDT
      mask TypeOptions OutMin: OutMin
      mask TypeOptions OutMax: OutMax
      mask TypeOptions OutDataTypeStr: OutDataTypeStr
      mask TypeOptions LockScale: LockScale
      mask TypeOptions RndMeth: RndMeth
      mask TypeOptions SaturateOnIntegerOverflow: SaturateOnIntegerOverflow
      mask DialogControl Container7 Prompt: メイン
      mask DialogControl Inputs Prompt: 入力数:
      mask DialogControl Multiplication Prompt: 乗算:
      mask DialogControl CollapseMode Prompt: 乗算範囲:
      mask DialogControl CollapseDim Prompt: 次元:
      mask DialogControl SampleTime Prompt: サンプル時間 (継承は -1):
      mask DialogControl Container8 Prompt: 信号属性
      mask DialogControl InputSameDT Prompt: すべての入力が同じデータ型をもつ
      mask DialogControl OutMin Prompt: 出力の最小値:
      mask DialogControl OutMax Prompt: 出力の最大値:
      mask DialogControl OutDataTypeStr Prompt: 出力データ型:
      mask DialogControl LockScale Prompt: 固定小数点ツールによる変更に対して出力データ型の設定をロックする
      mask DialogControl RndMeth Prompt: 整数丸めモード:
      mask DialogControl SaturateOnIntegerOverflow Prompt: 整数オーバーフローで飽和
  Function Caller : FunctionCaller  FunctionPrototype=[S15,U08] = J_get_vbc()  InputArgumentSpecifications=<Enter example>  OutputArgumentSpecifications=int16(ones(1,14)),uint8(1)
  Function Caller1 : FunctionCaller  FunctionPrototype=[S15,U08] = J_get_vbcmax()  InputArgumentSpecifications=<Enter example>  OutputArgumentSpecifications=int16(1),uint8(1)
  Function Caller10 : FunctionCaller  FunctionPrototype=[S31_1,U08,S31_2] = J_get_rbccaldmax()  InputArgumentSpecifications=<Enter example>  OutputArgumentSpecifications=int32(1),uint8(1),int32(1)
  Function Caller11 : FunctionCaller  FunctionPrototype=FLG1 = J_get_pwrofmd()  InputArgumentSpecifications=<Enter example>  OutputArgumentSpecifications=boolean(1)
  Function Caller12 : FunctionCaller  FunctionPrototype=[S15,U08] = J_get_vbcocvmax()  InputArgumentSpecifications=<Enter example>  OutputArgumentSpecifications=int16(1),uint8(1)
  Function Caller13 : FunctionCaller  FunctionPrototype=[U32,FLG] = J_get_tmbatoff()  InputArgumentSpecifications=<Enter example>  OutputArgumentSpecifications=uint32(1),boolean(1)
  Function Caller14 : FunctionCaller  FunctionPrototype=FLG = J_get_ocvmxninifn()  InputArgumentSpecifications=<Enter example>  OutputArgumentSpecifications=boolean(1)
  Function Caller15 : FunctionCaller  FunctionPrototype=[S15,U08] = J_get_vbcocvmin()  InputArgumentSpecifications=<Enter example>  OutputArgumentSpecifications=int16(1),uint8(1)
  Function Caller16 : FunctionCaller  FunctionPrototype=[sc_bcmax,st_scsoc] = J_get_scbcmax()  InputArgumentSpecifications=<Enter example>  OutputArgumentSpecifications=int16(1),uint8(1)
  Function Caller17 : FunctionCaller  FunctionPrototype=[sc_bcmin,st_scsoc] = J_get_scbcmin()  InputArgumentSpecifications=<Enter example>  OutputArgumentSpecifications=int16(1),uint8(1)
  Function Caller2 : FunctionCaller  FunctionPrototype=U16 = J_get_rbcrefini()  InputArgumentSpecifications=<Enter example>  OutputArgumentSpecifications=uint16(1)
  Function Caller3 : FunctionCaller  FunctionPrototype=[S15,U08] = J_get_tbmax()  InputArgumentSpecifications=<Enter example>  OutputArgumentSpecifications=int16(1),uint8(1)
  Function Caller4 : FunctionCaller  FunctionPrototype=[S15,U08] = J_get_tbmin()  InputArgumentSpecifications=<Enter example>  OutputArgumentSpecifications=int16(1),uint8(1)
  Function Caller5 : FunctionCaller  FunctionPrototype=[S15,U08] = J_get_ibat()  InputArgumentSpecifications=<Enter example>  OutputArgumentSpecifications=int16(1),uint8(1)
  Function Caller6 : FunctionCaller  FunctionPrototype=FLG = J_get_f_batuvmnt()  InputArgumentSpecifications=<Enter example>  OutputArgumentSpecifications=boolean(1)
  Function Caller7 : FunctionCaller  FunctionPrototype=[S31,U08] = J_get_asbcbasemin()  InputArgumentSpecifications=<Enter example>  OutputArgumentSpecifications=int32(1),uint8(1)
  Function Caller8 : FunctionCaller  FunctionPrototype=[U08_1,U08_2] = J_get_stimaop()  InputArgumentSpecifications=<Enter example>  OutputArgumentSpecifications=uint8(1),uint8(1)
  Function Caller9 : FunctionCaller  FunctionPrototype=[S31_1,U08,S31_2] = J_get_rbccalcmax()  InputArgumentSpecifications=<Enter example>  OutputArgumentSpecifications=int32(1),uint8(1),int32(1)
  LogicalOperator : Logic  Tag=#AMO_Lib  Inputs=Inputs  OutDataTypeStr=boolean  SampleTime=SampleTime  mask{Operator=AND, Inputs=2, IconShape=rectangular, SampleTime=-1, AllPortsSameDT=on, OutDataTypeStr=boolean}
      mask prompts: Operator "Simulink:blkprm_prompts:LogicOperator"; Inputs "Simulink:blkprm_prompts:LogicNumInputPorts"; IconShape "Simulink:blkprm_prompts:SumIconShape"; SampleTime "Simulink:blkprm_prompts:AllBlksSampleTime"; AllPortsSameDT "Simulink:blkprm_prompts:AllPortsSameDT"; OutDataTypeStr "Simulink:blkprm_prompts:OUTPUT_UNIFIEDDATATYPE"
      mask help: 論理演算です。単入力の場合、演算子は入力ベクトルに対して適用されます。多入力の場合、演算子は入力に対して適用されます。
      settings: AttributesFormatString=%<Tag>
      mask TypeOptions Operator: Operator
      mask TypeOptions Inputs: Inputs
      mask TypeOptions IconShape: IconShape
      mask TypeOptions SampleTime: SampleTime
      mask TypeOptions AllPortsSameDT: AllPortsSameDT
      mask TypeOptions OutDataTypeStr: OutDataTypeStr
      mask DialogControl Container4 Prompt: メイン
      mask DialogControl Operator Prompt: 演算子:
      mask DialogControl Inputs Prompt: 入力端子の数:
      mask DialogControl IconShape Prompt: アイコン形状:
      mask DialogControl SampleTime Prompt: サンプル時間 (継承は -1):
      mask DialogControl Container5 Prompt: データ型
      mask DialogControl AllPortsSameDT Prompt: すべての入出力が同じデータ型をもつ
      mask DialogControl OutDataTypeStr Prompt: 出力データ型:
  Model Header : Subsystem  mask(Model Header){ShowInLibBrowser=0}
      mask prompts: ShowInLibBrowser "Simulink:masks:CustCodeMaskParam1_MP"
      settings: CopyFcn=cccopyfcn(gcb)  OpenFcn=ccopenfcn('Model Header')
      mask Help: eval('feval(''rtwprivate'',''rtwhelpview'',''rtw_model_header_block'')');
      mask Display: disp('Model\nHeader');
  Model Source : Subsystem  mask(Model Source){ShowInLibBrowser=0}
      mask prompts: ShowInLibBrowser "Simulink:masks:CustCodeMaskParam1_MP"
      settings: CopyFcn=cccopyfcn(gcb)  OpenFcn=ccopenfcn('Model Source')
      mask Help: eval('feval(''rtwprivate'',''rtwhelpview'',''rtw_model_source_block'')');
      mask Display: disp('Model\nSource');
  RelationalOperator : RelationalOperator  Tag=#AMO_Lib  Operator===  OutDataTypeStr=boolean  SampleTime=SampleTime  RndMeth=Zero  InputSameDT=on  mask{Operator===, ZeroCross=on, SampleTime=-1, InputSameDT=on, OutDataTypeStr=boolean, RndMeth=Zero}
      mask prompts: Operator "Simulink:blkprm_prompts:RelopOperator"; ZeroCross "Simulink:blkprm_prompts:AllBlksEnableZC"; SampleTime "Simulink:blkprm_prompts:AllBlksSampleTime"; InputSameDT "Simulink:blkprm_prompts:InputSameDT"; OutDataTypeStr "Simulink:blkprm_prompts:OUTPUT_UNIFIEDDATATYPE"; RndMeth "Simulink:blkprm_prompts:SPP_RndMeth_ID"
      mask help: 入力に選択した関係演算子を適用し、結果を出力します。一番上 (または左） の入力は、最初のオペランドに対応します。
      settings: AttributesFormatString=%<Tag>
      mask TypeOptions Operator: Operator
      mask TypeOptions ZeroCross: ZeroCross
      mask TypeOptions SampleTime: SampleTime
      mask TypeOptions InputSameDT: InputSameDT
      mask TypeOptions OutDataTypeStr: OutDataTypeStr
      mask TypeOptions RndMeth: RndMeth
      mask DialogControl Container4 Prompt: メイン
      mask DialogControl Operator Prompt: 関係演算子:
      mask DialogControl ZeroCross Prompt: ゼロクロッシング検出を有効にする
      mask DialogControl SampleTime Prompt: サンプル時間 (継承は -1):
      mask DialogControl Container5 Prompt: データ型
      mask DialogControl InputSameDT Prompt: すべての入力が同じデータ型をもつ
      mask DialogControl OutDataTypeStr Prompt: 出力データ型:
      mask DialogControl RndMeth Prompt: 整数丸めモード:
  RelationalOperator1 : RelationalOperator  Tag=#AMO_Lib  Operator=<  OutDataTypeStr=boolean  SampleTime=SampleTime  RndMeth=Zero  InputSameDT=on  mask{Operator=<, ZeroCross=on, SampleTime=-1, InputSameDT=on, OutDataTypeStr=boolean, RndMeth=Zero}
      mask prompts: Operator "Simulink:blkprm_prompts:RelopOperator"; ZeroCross "Simulink:blkprm_prompts:AllBlksEnableZC"; SampleTime "Simulink:blkprm_prompts:AllBlksSampleTime"; InputSameDT "Simulink:blkprm_prompts:InputSameDT"; OutDataTypeStr "Simulink:blkprm_prompts:OUTPUT_UNIFIEDDATATYPE"; RndMeth "Simulink:blkprm_prompts:SPP_RndMeth_ID"
      mask help: 入力に選択した関係演算子を適用し、結果を出力します。一番上 (または左） の入力は、最初のオペランドに対応します。
      settings: AttributesFormatString=%<Tag>
      mask TypeOptions Operator: Operator
      mask TypeOptions ZeroCross: ZeroCross
      mask TypeOptions SampleTime: SampleTime
      mask TypeOptions InputSameDT: InputSameDT
      mask TypeOptions OutDataTypeStr: OutDataTypeStr
      mask TypeOptions RndMeth: RndMeth
      mask DialogControl Container4 Prompt: メイン
      mask DialogControl Operator Prompt: 関係演算子:
      mask DialogControl ZeroCross Prompt: ゼロクロッシング検出を有効にする
      mask DialogControl SampleTime Prompt: サンプル時間 (継承は -1):
      mask DialogControl Container5 Prompt: データ型
      mask DialogControl InputSameDT Prompt: すべての入力が同じデータ型をもつ
      mask DialogControl OutDataTypeStr Prompt: 出力データ型:
      mask DialogControl RndMeth Prompt: 整数丸めモード:
  Saturation : Saturate  Tag=#AMO_Lib  UpperLimit=UpperLimit  LowerLimit=LowerLimit  SampleTime=SampleTime  OutMin=OutMin  OutMax=OutMax  RndMeth=Zero  mask{UpperLimit=0.2, LowerLimit=0, LinearizeAsGain=on, ZeroCross=on, SampleTime=-1, OutMin=[], OutMax=[], OutDataTypeStr=Inherit: Same as input, LockScale=off, RndMeth=Zero}
      mask prompts: UpperLimit "Simulink:blkprm_prompts:SaturateUpLim"; LowerLimit "Simulink:blkprm_prompts:SaturateLowLim"; LinearizeAsGain "Simulink:blkprm_prompts:LinearizeAsGain"; ZeroCross "Simulink:blkprm_prompts:AllBlksEnableZC"; SampleTime "Simulink:blkprm_prompts:AllBlksSampleTime"; OutMin "Simulink:blkprm_prompts:OutputDesignMin"; OutMax "Simulink:blkprm_prompts:OutputDesignMax"; OutDataTypeStr "Simulink:blkprm_prompts:OUTPUT_UNIFIEDDATATYPE"; LockScale "Simulink:blkprm_prompts:LockScale"; RndMeth "Simulink:blkprm_prompts:SPP_RndMeth_ID"
      mask help: 入力信号を上限と下限の飽和値に制約します。
      settings: AttributesFormatString=%<Tag>\n%<LowerLimit> - %<UpperLimit>\nOutDataType = %<OutDataTypeStr>
      mask TypeOptions UpperLimit: UpperLimit
      mask TypeOptions LowerLimit: LowerLimit
      mask TypeOptions LinearizeAsGain: LinearizeAsGain
      mask TypeOptions ZeroCross: ZeroCross
      mask TypeOptions SampleTime: SampleTime
      mask TypeOptions OutMin: OutMin
      mask TypeOptions OutMax: OutMax
      mask TypeOptions OutDataTypeStr: OutDataTypeStr
      mask TypeOptions LockScale: LockScale
      mask TypeOptions RndMeth: RndMeth
      mask DialogControl Container4 Prompt: メイン
      mask DialogControl UpperLimit Prompt: 上限:
      mask DialogControl LowerLimit Prompt: 下限:
      mask DialogControl LinearizeAsGain Prompt: 線形化時にゲインとして扱う
      mask DialogControl ZeroCross Prompt: ゼロクロッシング検出を有効にする
      mask DialogControl SampleTime Prompt: サンプル時間 (継承は -1):
      mask DialogControl Container5 Prompt: 信号属性
      mask DialogControl OutMin Prompt: 出力の最小値:
      mask DialogControl OutMax Prompt: 出力の最大値:
      mask DialogControl OutDataTypeStr Prompt: 出力データ型:
      mask DialogControl LockScale Prompt: 固定小数点ツールによる変更に対して出力データ型の設定をロックする
      mask DialogControl RndMeth Prompt: 整数丸めモード:
  Saturation1 : Saturate  Tag=#AMO_Lib  UpperLimit=UpperLimit  LowerLimit=LowerLimit  SampleTime=SampleTime  OutMin=OutMin  OutMax=OutMax  RndMeth=Zero  mask{UpperLimit=100, LowerLimit=-100, LinearizeAsGain=on, ZeroCross=on, SampleTime=-1, OutMin=[], OutMax=[], OutDataTypeStr=Inherit: Same as input, LockScale=off, RndMeth=Zero}
      mask prompts: UpperLimit "Simulink:blkprm_prompts:SaturateUpLim"; LowerLimit "Simulink:blkprm_prompts:SaturateLowLim"; LinearizeAsGain "Simulink:blkprm_prompts:LinearizeAsGain"; ZeroCross "Simulink:blkprm_prompts:AllBlksEnableZC"; SampleTime "Simulink:blkprm_prompts:AllBlksSampleTime"; OutMin "Simulink:blkprm_prompts:OutputDesignMin"; OutMax "Simulink:blkprm_prompts:OutputDesignMax"; OutDataTypeStr "Simulink:blkprm_prompts:OUTPUT_UNIFIEDDATATYPE"; LockScale "Simulink:blkprm_prompts:LockScale"; RndMeth "Simulink:blkprm_prompts:SPP_RndMeth_ID"
      mask help: 入力信号を上限と下限の飽和値に制約します。
      settings: AttributesFormatString=%<Tag>\n%<LowerLimit> - %<UpperLimit>\nOutDataType = %<OutDataTypeStr>
      mask TypeOptions UpperLimit: UpperLimit
      mask TypeOptions LowerLimit: LowerLimit
      mask TypeOptions LinearizeAsGain: LinearizeAsGain
      mask TypeOptions ZeroCross: ZeroCross
      mask TypeOptions SampleTime: SampleTime
      mask TypeOptions OutMin: OutMin
      mask TypeOptions OutMax: OutMax
      mask TypeOptions OutDataTypeStr: OutDataTypeStr
      mask TypeOptions LockScale: LockScale
      mask TypeOptions RndMeth: RndMeth
      mask DialogControl Container4 Prompt: メイン
      mask DialogControl UpperLimit Prompt: 上限:
      mask DialogControl LowerLimit Prompt: 下限:
      mask DialogControl LinearizeAsGain Prompt: 線形化時にゲインとして扱う
      mask DialogControl ZeroCross Prompt: ゼロクロッシング検出を有効にする
      mask DialogControl SampleTime Prompt: サンプル時間 (継承は -1):
      mask DialogControl Container5 Prompt: 信号属性
      mask DialogControl OutMin Prompt: 出力の最小値:
      mask DialogControl OutMax Prompt: 出力の最大値:
      mask DialogControl OutDataTypeStr Prompt: 出力データ型:
      mask DialogControl LockScale Prompt: 固定小数点ツールによる変更に対して出力データ型の設定をロックする
      mask DialogControl RndMeth Prompt: 整数丸めモード:
  Saturation2 : Saturate  Tag=#AMO_Lib  UpperLimit=UpperLimit  LowerLimit=LowerLimit  SampleTime=SampleTime  OutMin=OutMin  OutMax=OutMax  RndMeth=Zero  mask{UpperLimit=100, LowerLimit=-100, LinearizeAsGain=on, ZeroCross=on, SampleTime=-1, OutMin=[], OutMax=[], OutDataTypeStr=Inherit: Same as input, LockScale=off, RndMeth=Zero}
      mask prompts: UpperLimit "Simulink:blkprm_prompts:SaturateUpLim"; LowerLimit "Simulink:blkprm_prompts:SaturateLowLim"; LinearizeAsGain "Simulink:blkprm_prompts:LinearizeAsGain"; ZeroCross "Simulink:blkprm_prompts:AllBlksEnableZC"; SampleTime "Simulink:blkprm_prompts:AllBlksSampleTime"; OutMin "Simulink:blkprm_prompts:OutputDesignMin"; OutMax "Simulink:blkprm_prompts:OutputDesignMax"; OutDataTypeStr "Simulink:blkprm_prompts:OUTPUT_UNIFIEDDATATYPE"; LockScale "Simulink:blkprm_prompts:LockScale"; RndMeth "Simulink:blkprm_prompts:SPP_RndMeth_ID"
      mask help: 入力信号を上限と下限の飽和値に制約します。
      settings: AttributesFormatString=%<Tag>\n%<LowerLimit> - %<UpperLimit>\nOutDataType = %<OutDataTypeStr>
      mask TypeOptions UpperLimit: UpperLimit
      mask TypeOptions LowerLimit: LowerLimit
      mask TypeOptions LinearizeAsGain: LinearizeAsGain
      mask TypeOptions ZeroCross: ZeroCross
      mask TypeOptions SampleTime: SampleTime
      mask TypeOptions OutMin: OutMin
      mask TypeOptions OutMax: OutMax
      mask TypeOptions OutDataTypeStr: OutDataTypeStr
      mask TypeOptions LockScale: LockScale
      mask TypeOptions RndMeth: RndMeth
      mask DialogControl Container4 Prompt: メイン
      mask DialogControl UpperLimit Prompt: 上限:
      mask DialogControl LowerLimit Prompt: 下限:
      mask DialogControl LinearizeAsGain Prompt: 線形化時にゲインとして扱う
      mask DialogControl ZeroCross Prompt: ゼロクロッシング検出を有効にする
      mask DialogControl SampleTime Prompt: サンプル時間 (継承は -1):
      mask DialogControl Container5 Prompt: 信号属性
      mask DialogControl OutMin Prompt: 出力の最小値:
      mask DialogControl OutMax Prompt: 出力の最大値:
      mask DialogControl OutDataTypeStr Prompt: 出力データ型:
      mask DialogControl LockScale Prompt: 固定小数点ツールによる変更に対して出力データ型の設定をロックする
      mask DialogControl RndMeth Prompt: 整数丸めモード:
  Saturation3 : Saturate  Tag=#AMO_Lib  UpperLimit=UpperLimit  LowerLimit=LowerLimit  SampleTime=SampleTime  OutMin=OutMin  OutMax=OutMax  RndMeth=Zero  mask{UpperLimit=360000, LowerLimit=0, LinearizeAsGain=on, ZeroCross=on, SampleTime=-1, OutMin=[], OutMax=[], OutDataTypeStr=Inherit: Same as input, LockScale=off, RndMeth=Zero}
      mask prompts: UpperLimit "Simulink:blkprm_prompts:SaturateUpLim"; LowerLimit "Simulink:blkprm_prompts:SaturateLowLim"; LinearizeAsGain "Simulink:blkprm_prompts:LinearizeAsGain"; ZeroCross "Simulink:blkprm_prompts:AllBlksEnableZC"; SampleTime "Simulink:blkprm_prompts:AllBlksSampleTime"; OutMin "Simulink:blkprm_prompts:OutputDesignMin"; OutMax "Simulink:blkprm_prompts:OutputDesignMax"; OutDataTypeStr "Simulink:blkprm_prompts:OUTPUT_UNIFIEDDATATYPE"; LockScale "Simulink:blkprm_prompts:LockScale"; RndMeth "Simulink:blkprm_prompts:SPP_RndMeth_ID"
      mask help: 入力信号を上限と下限の飽和値に制約します。
      settings: AttributesFormatString=%<Tag>\n%<LowerLimit> - %<UpperLimit>\nOutDataType = %<OutDataTypeStr>
      mask TypeOptions UpperLimit: UpperLimit
      mask TypeOptions LowerLimit: LowerLimit
      mask TypeOptions LinearizeAsGain: LinearizeAsGain
      mask TypeOptions ZeroCross: ZeroCross
      mask TypeOptions SampleTime: SampleTime
      mask TypeOptions OutMin: OutMin
      mask TypeOptions OutMax: OutMax
      mask TypeOptions OutDataTypeStr: OutDataTypeStr
      mask TypeOptions LockScale: LockScale
      mask TypeOptions RndMeth: RndMeth
      mask DialogControl Container4 Prompt: メイン
      mask DialogControl UpperLimit Prompt: 上限:
      mask DialogControl LowerLimit Prompt: 下限:
      mask DialogControl LinearizeAsGain Prompt: 線形化時にゲインとして扱う
      mask DialogControl ZeroCross Prompt: ゼロクロッシング検出を有効にする
      mask DialogControl SampleTime Prompt: サンプル時間 (継承は -1):
      mask DialogControl Container5 Prompt: 信号属性
      mask DialogControl OutMin Prompt: 出力の最小値:
      mask DialogControl OutMax Prompt: 出力の最大値:
      mask DialogControl OutDataTypeStr Prompt: 出力データ型:
      mask DialogControl LockScale Prompt: 固定小数点ツールによる変更に対して出力データ型の設定をロックする
      mask DialogControl RndMeth Prompt: 整数丸めモード:
  Saturation4 : Saturate  Tag=#AMO_Lib  UpperLimit=UpperLimit  LowerLimit=LowerLimit  SampleTime=SampleTime  OutMin=OutMin  OutMax=OutMax  RndMeth=Zero  mask{UpperLimit=100, LowerLimit=0, LinearizeAsGain=on, ZeroCross=on, SampleTime=-1, OutMin=[], OutMax=[], OutDataTypeStr=Inherit: Same as input, LockScale=off, RndMeth=Zero}
      mask prompts: UpperLimit "Simulink:blkprm_prompts:SaturateUpLim"; LowerLimit "Simulink:blkprm_prompts:SaturateLowLim"; LinearizeAsGain "Simulink:blkprm_prompts:LinearizeAsGain"; ZeroCross "Simulink:blkprm_prompts:AllBlksEnableZC"; SampleTime "Simulink:blkprm_prompts:AllBlksSampleTime"; OutMin "Simulink:blkprm_prompts:OutputDesignMin"; OutMax "Simulink:blkprm_prompts:OutputDesignMax"; OutDataTypeStr "Simulink:blkprm_prompts:OUTPUT_UNIFIEDDATATYPE"; LockScale "Simulink:blkprm_prompts:LockScale"; RndMeth "Simulink:blkprm_prompts:SPP_RndMeth_ID"
      mask help: 入力信号を上限と下限の飽和値に制約します。
      settings: AttributesFormatString=%<Tag>\n%<LowerLimit> - %<UpperLimit>\nOutDataType = %<OutDataTypeStr>
      mask TypeOptions UpperLimit: UpperLimit
      mask TypeOptions LowerLimit: LowerLimit
      mask TypeOptions LinearizeAsGain: LinearizeAsGain
      mask TypeOptions ZeroCross: ZeroCross
      mask TypeOptions SampleTime: SampleTime
      mask TypeOptions OutMin: OutMin
      mask TypeOptions OutMax: OutMax
      mask TypeOptions OutDataTypeStr: OutDataTypeStr
      mask TypeOptions LockScale: LockScale
      mask TypeOptions RndMeth: RndMeth
      mask DialogControl Container4 Prompt: メイン
      mask DialogControl UpperLimit Prompt: 上限:
      mask DialogControl LowerLimit Prompt: 下限:
      mask DialogControl LinearizeAsGain Prompt: 線形化時にゲインとして扱う
      mask DialogControl ZeroCross Prompt: ゼロクロッシング検出を有効にする
      mask DialogControl SampleTime Prompt: サンプル時間 (継承は -1):
      mask DialogControl Container5 Prompt: 信号属性
      mask DialogControl OutMin Prompt: 出力の最小値:
      mask DialogControl OutMax Prompt: 出力の最大値:
      mask DialogControl OutDataTypeStr Prompt: 出力データ型:
      mask DialogControl LockScale Prompt: 固定小数点ツールによる変更に対して出力データ型の設定をロックする
      mask DialogControl RndMeth Prompt: 整数丸めモード:
  Saturation5 : Saturate  Tag=#AMO_Lib  UpperLimit=UpperLimit  LowerLimit=LowerLimit  SampleTime=SampleTime  OutMin=OutMin  OutMax=OutMax  RndMeth=Zero  mask{UpperLimit=10, LowerLimit=-10, LinearizeAsGain=on, ZeroCross=on, SampleTime=-1, OutMin=[], OutMax=[], OutDataTypeStr=Inherit: Same as input, LockScale=off, RndMeth=Zero}
      mask prompts: UpperLimit "Simulink:blkprm_prompts:SaturateUpLim"; LowerLimit "Simulink:blkprm_prompts:SaturateLowLim"; LinearizeAsGain "Simulink:blkprm_prompts:LinearizeAsGain"; ZeroCross "Simulink:blkprm_prompts:AllBlksEnableZC"; SampleTime "Simulink:blkprm_prompts:AllBlksSampleTime"; OutMin "Simulink:blkprm_prompts:OutputDesignMin"; OutMax "Simulink:blkprm_prompts:OutputDesignMax"; OutDataTypeStr "Simulink:blkprm_prompts:OUTPUT_UNIFIEDDATATYPE"; LockScale "Simulink:blkprm_prompts:LockScale"; RndMeth "Simulink:blkprm_prompts:SPP_RndMeth_ID"
      mask help: 入力信号を上限と下限の飽和値に制約します。
      settings: AttributesFormatString=%<Tag>\n%<LowerLimit> - %<UpperLimit>\nOutDataType = %<OutDataTypeStr>
      mask TypeOptions UpperLimit: UpperLimit
      mask TypeOptions LowerLimit: LowerLimit
      mask TypeOptions LinearizeAsGain: LinearizeAsGain
      mask TypeOptions ZeroCross: ZeroCross
      mask TypeOptions SampleTime: SampleTime
      mask TypeOptions OutMin: OutMin
      mask TypeOptions OutMax: OutMax
      mask TypeOptions OutDataTypeStr: OutDataTypeStr
      mask TypeOptions LockScale: LockScale
      mask TypeOptions RndMeth: RndMeth
      mask DialogControl Container4 Prompt: メイン
      mask DialogControl UpperLimit Prompt: 上限:
      mask DialogControl LowerLimit Prompt: 下限:
      mask DialogControl LinearizeAsGain Prompt: 線形化時にゲインとして扱う
      mask DialogControl ZeroCross Prompt: ゼロクロッシング検出を有効にする
      mask DialogControl SampleTime Prompt: サンプル時間 (継承は -1):
      mask DialogControl Container5 Prompt: 信号属性
      mask DialogControl OutMin Prompt: 出力の最小値:
      mask DialogControl OutMax Prompt: 出力の最大値:
      mask DialogControl OutDataTypeStr Prompt: 出力データ型:
      mask DialogControl LockScale Prompt: 固定小数点ツールによる変更に対して出力データ型の設定をロックする
      mask DialogControl RndMeth Prompt: 整数丸めモード:
  Saturation6 : Saturate  Tag=#AMO_Lib  UpperLimit=UpperLimit  LowerLimit=LowerLimit  SampleTime=SampleTime  OutMin=OutMin  OutMax=OutMax  RndMeth=Zero  mask{UpperLimit=10, LowerLimit=-10, LinearizeAsGain=on, ZeroCross=on, SampleTime=-1, OutMin=[], OutMax=[], OutDataTypeStr=Inherit: Same as input, LockScale=off, RndMeth=Zero}
      mask prompts: UpperLimit "Simulink:blkprm_prompts:SaturateUpLim"; LowerLimit "Simulink:blkprm_prompts:SaturateLowLim"; LinearizeAsGain "Simulink:blkprm_prompts:LinearizeAsGain"; ZeroCross "Simulink:blkprm_prompts:AllBlksEnableZC"; SampleTime "Simulink:blkprm_prompts:AllBlksSampleTime"; OutMin "Simulink:blkprm_prompts:OutputDesignMin"; OutMax "Simulink:blkprm_prompts:OutputDesignMax"; OutDataTypeStr "Simulink:blkprm_prompts:OUTPUT_UNIFIEDDATATYPE"; LockScale "Simulink:blkprm_prompts:LockScale"; RndMeth "Simulink:blkprm_prompts:SPP_RndMeth_ID"
      mask help: 入力信号を上限と下限の飽和値に制約します。
      settings: AttributesFormatString=%<Tag>\n%<LowerLimit> - %<UpperLimit>\nOutDataType = %<OutDataTypeStr>
      mask TypeOptions UpperLimit: UpperLimit
      mask TypeOptions LowerLimit: LowerLimit
      mask TypeOptions LinearizeAsGain: LinearizeAsGain
      mask TypeOptions ZeroCross: ZeroCross
      mask TypeOptions SampleTime: SampleTime
      mask TypeOptions OutMin: OutMin
      mask TypeOptions OutMax: OutMax
      mask TypeOptions OutDataTypeStr: OutDataTypeStr
      mask TypeOptions LockScale: LockScale
      mask TypeOptions RndMeth: RndMeth
      mask DialogControl Container4 Prompt: メイン
      mask DialogControl UpperLimit Prompt: 上限:
      mask DialogControl LowerLimit Prompt: 下限:
      mask DialogControl LinearizeAsGain Prompt: 線形化時にゲインとして扱う
      mask DialogControl ZeroCross Prompt: ゼロクロッシング検出を有効にする
      mask DialogControl SampleTime Prompt: サンプル時間 (継承は -1):
      mask DialogControl Container5 Prompt: 信号属性
      mask DialogControl OutMin Prompt: 出力の最小値:
      mask DialogControl OutMax Prompt: 出力の最大値:
      mask DialogControl OutDataTypeStr Prompt: 出力データ型:
      mask DialogControl LockScale Prompt: 固定小数点ツールによる変更に対して出力データ型の設定をロックする
      mask DialogControl RndMeth Prompt: 整数丸めモード:
  Saturation7 : Saturate  Tag=#AMO_Lib  UpperLimit=UpperLimit  LowerLimit=LowerLimit  SampleTime=SampleTime  OutMin=OutMin  OutMax=OutMax  RndMeth=Zero  mask{UpperLimit=100, LowerLimit=-100, LinearizeAsGain=on, ZeroCross=on, SampleTime=-1, OutMin=[], OutMax=[], OutDataTypeStr=Inherit: Same as input, LockScale=off, RndMeth=Zero}
      mask prompts: UpperLimit "Simulink:blkprm_prompts:SaturateUpLim"; LowerLimit "Simulink:blkprm_prompts:SaturateLowLim"; LinearizeAsGain "Simulink:blkprm_prompts:LinearizeAsGain"; ZeroCross "Simulink:blkprm_prompts:AllBlksEnableZC"; SampleTime "Simulink:blkprm_prompts:AllBlksSampleTime"; OutMin "Simulink:blkprm_prompts:OutputDesignMin"; OutMax "Simulink:blkprm_prompts:OutputDesignMax"; OutDataTypeStr "Simulink:blkprm_prompts:OUTPUT_UNIFIEDDATATYPE"; LockScale "Simulink:blkprm_prompts:LockScale"; RndMeth "Simulink:blkprm_prompts:SPP_RndMeth_ID"
      mask help: 入力信号を上限と下限の飽和値に制約します。
      settings: AttributesFormatString=%<Tag>\n%<LowerLimit> - %<UpperLimit>\nOutDataType = %<OutDataTypeStr>
      mask TypeOptions UpperLimit: UpperLimit
      mask TypeOptions LowerLimit: LowerLimit
      mask TypeOptions LinearizeAsGain: LinearizeAsGain
      mask TypeOptions ZeroCross: ZeroCross
      mask TypeOptions SampleTime: SampleTime
      mask TypeOptions OutMin: OutMin
      mask TypeOptions OutMax: OutMax
      mask TypeOptions OutDataTypeStr: OutDataTypeStr
      mask TypeOptions LockScale: LockScale
      mask TypeOptions RndMeth: RndMeth
      mask DialogControl Container4 Prompt: メイン
      mask DialogControl UpperLimit Prompt: 上限:
      mask DialogControl LowerLimit Prompt: 下限:
      mask DialogControl LinearizeAsGain Prompt: 線形化時にゲインとして扱う
      mask DialogControl ZeroCross Prompt: ゼロクロッシング検出を有効にする
      mask DialogControl SampleTime Prompt: サンプル時間 (継承は -1):
      mask DialogControl Container5 Prompt: 信号属性
      mask DialogControl OutMin Prompt: 出力の最小値:
      mask DialogControl OutMax Prompt: 出力の最大値:
      mask DialogControl OutDataTypeStr Prompt: 出力データ型:
      mask DialogControl LockScale Prompt: 固定小数点ツールによる変更に対して出力データ型の設定をロックする
      mask DialogControl RndMeth Prompt: 整数丸めモード:
  Saturation8 : Saturate  Tag=#AMO_Lib  UpperLimit=UpperLimit  LowerLimit=LowerLimit  SampleTime=SampleTime  OutMin=OutMin  OutMax=OutMax  RndMeth=Zero  mask{UpperLimit=100, LowerLimit=-100, LinearizeAsGain=on, ZeroCross=on, SampleTime=-1, OutMin=[], OutMax=[], OutDataTypeStr=Inherit: Same as input, LockScale=off, RndMeth=Zero}
      mask prompts: UpperLimit "Simulink:blkprm_prompts:SaturateUpLim"; LowerLimit "Simulink:blkprm_prompts:SaturateLowLim"; LinearizeAsGain "Simulink:blkprm_prompts:LinearizeAsGain"; ZeroCross "Simulink:blkprm_prompts:AllBlksEnableZC"; SampleTime "Simulink:blkprm_prompts:AllBlksSampleTime"; OutMin "Simulink:blkprm_prompts:OutputDesignMin"; OutMax "Simulink:blkprm_prompts:OutputDesignMax"; OutDataTypeStr "Simulink:blkprm_prompts:OUTPUT_UNIFIEDDATATYPE"; LockScale "Simulink:blkprm_prompts:LockScale"; RndMeth "Simulink:blkprm_prompts:SPP_RndMeth_ID"
      mask help: 入力信号を上限と下限の飽和値に制約します。
      settings: AttributesFormatString=%<Tag>\n%<LowerLimit> - %<UpperLimit>\nOutDataType = %<OutDataTypeStr>
      mask TypeOptions UpperLimit: UpperLimit
      mask TypeOptions LowerLimit: LowerLimit
      mask TypeOptions LinearizeAsGain: LinearizeAsGain
      mask TypeOptions ZeroCross: ZeroCross
      mask TypeOptions SampleTime: SampleTime
      mask TypeOptions OutMin: OutMin
      mask TypeOptions OutMax: OutMax
      mask TypeOptions OutDataTypeStr: OutDataTypeStr
      mask TypeOptions LockScale: LockScale
      mask TypeOptions RndMeth: RndMeth
      mask DialogControl Container4 Prompt: メイン
      mask DialogControl UpperLimit Prompt: 上限:
      mask DialogControl LowerLimit Prompt: 下限:
      mask DialogControl LinearizeAsGain Prompt: 線形化時にゲインとして扱う
      mask DialogControl ZeroCross Prompt: ゼロクロッシング検出を有効にする
      mask DialogControl SampleTime Prompt: サンプル時間 (継承は -1):
      mask DialogControl Container5 Prompt: 信号属性
      mask DialogControl OutMin Prompt: 出力の最小値:
      mask DialogControl OutMax Prompt: 出力の最大値:
      mask DialogControl OutDataTypeStr Prompt: 出力データ型:
      mask DialogControl LockScale Prompt: 固定小数点ツールによる変更に対して出力データ型の設定をロックする
      mask DialogControl RndMeth Prompt: 整数丸めモード:
  Subsystem : Subsystem
  System Outputs : Subsystem  mask(System Outputs){ShowInLibBrowser=0}
      mask prompts: ShowInLibBrowser "Simulink:masks:CustCodeMaskParam1_MP"
      settings: CopyFcn=cccopyfcn(gcb)  OpenFcn=ccopenfcn('System Outputs Function')
      mask Help: eval('feval(''rtwprivate'',''rtwhelpview'',''rtw_sys_outputs_block'')');
      mask Display: disp('System\nOutputs');
  System Update : Subsystem  mask(System Update){ShowInLibBrowser=0}
      mask prompts: ShowInLibBrowser "Simulink:masks:CustCodeMaskParam1_MP"
      settings: CopyFcn=cccopyfcn(gcb)  OpenFcn=ccopenfcn('System Update Function')
      mask Help: eval('feval(''rtwprivate'',''rtwhelpview'',''rtw_sys_update_block'')');
      mask Display: disp('System\nUpdate');
  Terminator{,1..10} (11 alike) : Terminator
      settings: Tag=#AMO_Lib  AttributesFormatString=%<Tag>
  Unit Delay : UnitDelay  Tag=#AMO_Lib  SampleTime=-1  HasFrameUpgradeWarning=on
      settings: AttributesFormatString=%<Tag>\nInitialCondition = %<InitialCondition>\nSampleTime = %<SampleTime>
  stopengstmode_C : Constant  Tag=#AMO_Lib  Value=stopengstmode_C
      settings: AttributesFormatString=%<Tag>\nOutDataType = %<OutDataTypeStr>
  t_vminddstr_C : Constant  Tag=#AMO_Lib  Value=t_vminddstr_C
      settings: AttributesFormatString=%<Tag>\nOutDataType = %<OutDataTypeStr>
  v_bc_pl_s : Outport  Tag=#AMO_Lib  InitialOutput=0
      settings: AttributesFormatString=%<Tag>\n%<Description>\nInitialOutput = %<InitialOutput>
  st_vbc_pl : Outport  Tag=#AMO_Lib  Port=2  InitialOutput=0
      settings: AttributesFormatString=%<Tag>\n%<Description>\nInitialOutput = %<InitialOutput>
  r_estd_ini_s : Outport  Tag=#AMO_Lib  Port=3  InitialOutput=0
      settings: AttributesFormatString=%<Tag>\n%<Description>\nInitialOutput = %<InitialOutput>
  r_estc_ini_s : Outport  Tag=#AMO_Lib  Port=4  InitialOutput=0
      settings: AttributesFormatString=%<Tag>\n%<Description>\nInitialOutput = %<InitialOutput>
  t_bmax_pl_s : Outport  Tag=#AMO_Lib  Port=5  InitialOutput=0
      settings: AttributesFormatString=%<Tag>\n%<Description>\nInitialOutput = %<InitialOutput>
  st_tbmax_pl : Outport  Tag=#AMO_Lib  Port=6  InitialOutput=0
      settings: AttributesFormatString=%<Tag>\n%<Description>\nInitialOutput = %<InitialOutput>
  t_bmin_pl_s : Outport  Tag=#AMO_Lib  Port=7  InitialOutput=0
      settings: AttributesFormatString=%<Tag>\n%<Description>\nInitialOutput = %<InitialOutput>
  st_tbmin_pl : Outport  Tag=#AMO_Lib  Port=8  InitialOutput=0
      settings: AttributesFormatString=%<Tag>\n%<Description>\nInitialOutput = %<InitialOutput>
  as_bcbsmin_pl_s : Outport  Tag=#AMO_Lib  Port=9  InitialOutput=0
      settings: AttributesFormatString=%<Tag>\n%<Description>\nInitialOutput = %<InitialOutput>
  i_bat_10m_pl : Outport  Tag=#AMO_Lib  Port=10  InitialOutput=0
      settings: AttributesFormatString=%<Tag>\n%<Description>\nInitialOutput = %<InitialOutput>
  i_bat_10m_pl_s : Outport  Tag=#AMO_Lib  Port=11  InitialOutput=0
      settings: AttributesFormatString=%<Tag>\n%<Description>\nInitialOutput = %<InitialOutput>
  st_ibat_10m_pl : Outport  Tag=#AMO_Lib  Port=12  InitialOutput=0
      settings: AttributesFormatString=%<Tag>\n%<Description>\nInitialOutput = %<InitialOutput>
  iwboxcdf_pl_s : Outport  Tag=#AMO_Lib  Port=13  InitialOutput=0
      settings: AttributesFormatString=%<Tag>\n%<Description>\nInitialOutput = %<InitialOutput>
  v_bcocvmax_pl_s : Outport  Tag=#AMO_Lib  Port=14  InitialOutput=0
      settings: AttributesFormatString=%<Tag>\n%<Description>\nInitialOutput = %<InitialOutput>
  v_bcocvmin_pl_s : Outport  Tag=#AMO_Lib  Port=15  InitialOutput=0
      settings: AttributesFormatString=%<Tag>\n%<Description>\nInitialOutput = %<InitialOutput>
  f_pwexprq : Outport  Tag=#AMO_Lib  Port=16  InitialOutput=0
      settings: AttributesFormatString=%<Tag>\n%<Description>\nInitialOutput = %<InitialOutput>
  f_batuvmnt_pl : Outport  Tag=#AMO_Lib  Port=17  InitialOutput=0
      settings: AttributesFormatString=%<Tag>\n%<Description>\nInitialOutput = %<InitialOutput>
  krcadj_pl_s : Outport  Tag=#AMO_Lib  Port=18  InitialOutput=0
      settings: AttributesFormatString=%<Tag>\n%<Description>\nInitialOutput = %<InitialOutput>
  krdadj_pl_s : Outport  Tag=#AMO_Lib  Port=19  InitialOutput=0
      settings: AttributesFormatString=%<Tag>\n%<Description>\nInitialOutput = %<InitialOutput>
  f_pwrofmdhv_pl : Outport  Tag=#AMO_Lib  Port=20  InitialOutput=0
      settings: AttributesFormatString=%<Tag>\n%<Description>\nInitialOutput = %<InitialOutput>
  tmbatoff_pl : Outport  Tag=#AMO_Lib  Port=21  InitialOutput=0
      settings: AttributesFormatString=%<Tag>\n%<Description>\nInitialOutput = %<InitialOutput>
  f_tmbatoffn_pl : Outport  Tag=#AMO_Lib  Port=22  InitialOutput=0
      settings: AttributesFormatString=%<Tag>\n%<Description>\nInitialOutput = %<InitialOutput>
  v_bcmax_pl : Outport  Tag=#AMO_Lib  Port=23  InitialOutput=0
      settings: AttributesFormatString=%<Tag>\n%<Description>\nInitialOutput = %<InitialOutput>
  f_ocvmxninifn_pl : Outport  Tag=#AMO_Lib  Port=24  InitialOutput=0
      settings: AttributesFormatString=%<Tag>\n%<Description>\nInitialOutput = %<InitialOutput>
  sc_bcmax_pl : Outport  Tag=#AMO_Lib  Port=25  InitialOutput=0
      settings: AttributesFormatString=%<Tag>\n%<Description>\nInitialOutput = %<InitialOutput>
  sc_bcmin_pl : Outport  Tag=#AMO_Lib  Port=26  InitialOutput=0
      settings: AttributesFormatString=%<Tag>\n%<Description>\nInitialOutput = %<InitialOutput>
  wires:
  Function Caller/2 -> st_vbc_pl/1
  Function Caller/1 -> Data Type Conversion/1
  Constant/1 -> Divide/2
  Data Type Conversion/1 -> Divide/1
  Divide/1 -> Data Type Conversion30/1
  Function Caller2/1 -> Data Type Conversion1/1
  Data Type Conversion1/1 -> Divide1/1
  Constant1/1 -> Divide1/2
  Divide1/1 -> Data Type Conversion2/1
  Saturation/1 -> r_estc_ini_s/1, r_estd_ini_s/1
  Data Type Conversion2/1 -> Saturation/1
  Data Type Conversion3/1 -> Divide2/1
  Constant2/1 -> Divide2/2
  Divide2/1 -> Data Type Conversion4/1
  Function Caller3/1 -> Data Type Conversion3/1
  Data Type Conversion4/1 -> Saturation1/1
  Saturation1/1 -> t_bmax_pl_s/1
  Function Caller3/2 -> st_tbmax_pl/1
  Constant3/1 -> Divide3/2
  Function Caller4/2 -> st_tbmin_pl/1
  Divide3/1 -> Data Type Conversion6/1
  Data Type Conversion5/1 -> Divide3/1
  Data Type Conversion6/1 -> Saturation2/1
  Saturation2/1 -> t_bmin_pl_s/1
  Function Caller4/1 -> Data Type Conversion17/1, Data Type Conversion5/1
  Data Type Conversion8/1 -> Saturation3/1
  Function Caller7/2 -> Terminator/1
  Saturation3/1 -> as_bcbsmin_pl_s/1
  Divide4/1 -> Data Type Conversion8/1
  Data Type Conversion7/1 -> Divide4/1
  Constant4/1 -> Divide4/2
  Function Caller7/1 -> Data Type Conversion7/1
  Function Caller5/1 -> Subsystem/1(i_bat)
  Function Caller5/2 -> Subsystem/2(st_ibat), st_ibat_10m_pl/1
  Z_i_bat_10m_pl/1 -> Subsystem/3(Z_i_bat_10m_pl)
  Subsystem/2(i_bat_10m_pll) -> Unit Delay/1
  Unit Delay/1 -> Subsystem/4(Z_i_bat_10m_pll)
  Divide5/1 -> Data Type Conversion11/1
  Constant5/1 -> Divide5/2
  Data Type Conversion10/1 -> Divide5/1
  Data Type Conversion11/1 -> i_bat_10m_pl_s/1
  Divide6/1 -> Data Type Conversion12/1
  Data Type Conversion12/1 -> Saturation4/1
  Constant6/1 -> Divide6/2
  Data Type Conversion9/1 -> Divide6/1
  Saturation4/1 -> iwboxcdf_pl_s/1
  Saturation5/1 -> v_bcocvmax_pl_s/1
  Data Type Conversion13/1 -> Saturation5/1
  Data Type Conversion14/1 -> Divide7/1
  Divide7/1 -> Data Type Conversion13/1
  Constant7/1 -> Divide7/2
  Function Caller12/1 -> Data Type Conversion14/1
  Function Caller15/2 -> Terminator1/1
  Divide8/1 -> Data Type Conversion16/1
  Data Type Conversion16/1 -> Saturation6/1
  Constant8/1 -> Divide8/2
  Function Caller15/1 -> Data Type Conversion15/1
  Data Type Conversion15/1 -> Divide8/1
  Saturation6/1 -> v_bcocvmin_pl_s/1
  Function Caller12/2 -> Terminator2/1
  Data Type Conversion17/1 -> [t_bmin]
  RelationalOperator/1 -> LogicalOperator/1
  Function Caller8/1 -> RelationalOperator/1
  stopengstmode_C/1 -> RelationalOperator/2
  RelationalOperator1/1 -> LogicalOperator/2
  t_vminddstr_C/1 -> RelationalOperator1/2
  [t_bmin] -> RelationalOperator1/1
  LogicalOperator/1 -> f_pwexprq/1
  Function Caller6/1 -> Data Type Conversion29/1
  Function Caller9/1 -> Terminator3/1
  Divide9/1 -> Data Type Conversion19/1
  Constant9/1 -> Divide9/2
  Data Type Conversion18/1 -> Divide9/1
  Function Caller9/3 -> Data Type Conversion18/1
  Data Type Conversion19/1 -> Saturation7/1
  Saturation7/1 -> krcadj_pl_s/1
  Function Caller9/2 -> Terminator4/1
  Saturation8/1 -> krdadj_pl_s/1
  Function Caller10/3 -> Data Type Conversion20/1
  Data Type Conversion21/1 -> Saturation8/1
  Constant10/1 -> Divide10/2
  Function Caller10/1 -> Terminator5/1
  Divide10/1 -> Data Type Conversion21/1
  Data Type Conversion20/1 -> Divide10/1
  Function Caller10/2 -> Terminator6/1
  Function Caller11/1 -> Data Type Conversion22/1
  Function Caller1/1 -> Data Type Conversion25/1
  Data Type Conversion22/1 -> f_pwrofmdhv_pl/1
  Function Caller13/1 -> Data Type Conversion23/1
  Function Caller13/2 -> Data Type Conversion24/1
  Data Type Conversion25/1 -> v_bcmax_pl/1
  Data Type Conversion23/1 -> tmbatoff_pl/1
  Data Type Conversion24/1 -> f_tmbatoffn_pl/1
  Function Caller1/2 -> Terminator7/1
  Function Caller14/1 -> Data Type Conversion26/1
  Data Type Conversion26/1 -> f_ocvmxninifn_pl/1
  Function Caller16/2 -> Terminator8/1
  Function Caller16/1 -> Data Type Conversion27/1
  Data Type Conversion27/1 -> sc_bcmax_pl/1
  Data Type Conversion28/1 -> sc_bcmin_pl/1
  Function Caller17/1 -> Data Type Conversion28/1
  Function Caller17/2 -> Terminator9/1
  Data Type Conversion29/1 -> f_batuvmnt_pl/1
  Data Type Conversion30/1 -> v_bc_pl_s/1
  Subsystem/1(i_bat_10m_pl) -> i_bat_10m_pl/1, Data Type Conversion10/1
  Function Caller8/2 -> Terminator10/1
  iwboxcdf/1 -> Data Type Conversion9/1
